simulink library "ammclib_bam_S32K3xx"  (R2016a)
(part 4 of 50)

      |     warning(['Parameter f16PropGain_Q of ' gcb ' exceeds the fixed-point range.']);
      |   end
      |   if f16PropGain_Q<-2^15
      |     f16PropGain_Q=-2^15;
      |     warning(['Parameter f16PropGain_Q of ' gcb ' exceeds the fixed-point range.']);
      |   end
      |   kifQ=igainQ*SampleTime*0.5*iscale/uscale;
      |   s16IntegGainShift_Q=ceil(log2(abs(kifQ)));
      |   if s16IntegGainShift_Q<-15
      |     s16IntegGainShift_Q=-15;
      |   end
      |   if s16IntegGainShift_Q>15
      |     s16IntegGainShift_Q=15;
      |     warning(['Parameter s16IntegGainShift_Q of ' gcb ' exceeds the fixed-point range.']);
      |   end
      |   f16IntegGain_Q=round(kifQ*2^(-s16IntegGainShift_Q)*2^15);
      |   if f16IntegGain_Q>2^15-1
      |     f16IntegGain_Q=2^15-1;
      |     warning(['Parameter f16IntegGain_Q of ' gcb ' exceeds the fixed-point range.']);
      |   end
      |   if f16IntegGain_Q<-2^15
      |     f16IntegGain_Q=-2^15;
      |     warning(['Parameter f16IntegGain_Q of ' gcb ' exceeds the fixed-point range.']);
      |   end
      |   if isnan(f16PropGain_D)
      |     if ~strcmp(f16PropGain_D_bkup,'0')
      |       set_param(gcb,'f16PropGain_D','0');
      |     end
      |   else
      |     tmps=num2str(f16PropGain_D);
      |     if ~strcmp(f16PropGain_D_bkup,tmps)
      |       set_param(gcb,'f16PropGain_D',tmps);
      |     end
      |   end
      |   if isnan(f16IntegGain_D)
      |     if ~strcmp(f16IntegGain_D_bkup,'0')
      |       set_param(gcb,'f16IntegGain_D','0');
      |     end
      |   else
      |     tmps=num2str(f16IntegGain_D);
      |     if ~strcmp(f16IntegGain_D_bkup,tmps)
      |       set_param(gcb,'f16IntegGain_D',tmps);
      |     end
      |   end
      |   if isnan(s16PropGainShift_D)
      |     if ~strcmp(s16PropGainShift_D_bkup,'0')
      |       set_param(gcb,'s16PropGainShift_D','0');
      |     end
      |   else
      |     tmps=num2str(s16PropGainShift_D);
      |     if ~strcmp(s16PropGainShift_D_bkup,tmps)
      |       set_param(gcb,'s16PropGainShift_D',tmps);
      |     end
      |   end
      |   if isnan(s16IntegGainShift_D)
      |     if ~strcmp(s16IntegGainShift_D_bkup,'0')
      |       set_param(gcb,'s16IntegGainShift_D','0');
      |     end
      |   else
      |     tmps=num2str(s16IntegGainShift_D);
      |     if ~strcmp(s16IntegGainShift_D_bkup,tmps)
      |       set_param(gcb,'s16IntegGainShift_D',tmps);
      |     end
      |   end
      |   if isnan(f16PropGain_Q)
      |     if ~strcmp(f16PropGain_Q_bkup,'0')
      |       set_param(gcb,'f16PropGain_Q','0');
      |     end
      |   else
      |     tmps=num2str(f16PropGain_Q);
      |     if ~strcmp(f16PropGain_Q_bkup,tmps)
      |       set_param(gcb,'f16PropGain_Q',tmps);
      |     end
      |   end
      |   if isnan(f16IntegGain_Q)
      |     if ~strcmp(f16IntegGain_Q_bkup,'0')
      |       set_param(gcb,'f16IntegGain_Q','0');
      |     end
      |   else
      |     tmps=num2str(f16IntegGain_Q);
      |     if ~strcmp(f16IntegGain_Q_bkup,tmps)
      |       set_param(gcb,'f16IntegGain_Q',tmps);
      |     end
      |   end
      |   if isnan(s16PropGainShift_Q)
      |     if ~strcmp(s16PropGainShift_Q_bkup,'0')
      |       set_param(gcb,'s16PropGainShift_Q','0');
      |     end
      |   else
      |     tmps=num2str(s16PropGainShift_Q);
      |     if ~strcmp(s16PropGainShift_Q_bkup,tmps)
      |       set_param(gcb,'s16PropGainShift_Q',tmps);
      |     end
      |   end
      |   if isnan(s16IntegGainShift_Q)
      |     if ~strcmp(s16IntegGainShift_Q_bkup,'0')
      |       set_param(gcb,'s16IntegGainShift_Q','0');
      |     end
      |   else
      |     tmps=num2str(s16IntegGainShift_Q);
      |     if ~strcmp(s16IntegGainShift_Q_bkup,tmps)
      |       set_param(gcb,'s16IntegGainShift_Q',tmps);
      |     end
      |   end
      | end
      mask Callback Lq:
      | autoCalcEn=get_param(gcb,'autoCalcEn');
      | if strcmp(autoCalcEn,'on')
      |   SampleTime=Simulink.data.evalinGlobal(bdroot,get_param(gcb,'SampleTime'));
      |   if (SampleTime==-1)
      |     SampleTime=str2double(get_param(gcb,'SampleTime_1'));
      |   end
      |   f16PropGain_D_bkup=get_param(gcb,'f16PropGain_D');
      |   f16IntegGain_D_bkup=get_param(gcb,'f16IntegGain_D');
      |   s16PropGainShift_D_bkup=get_param(gcb,'s16PropGainShift_D');
      |   s16IntegGainShift_D_bkup=get_param(gcb,'s16IntegGainShift_D');
      |   f16PropGain_Q_bkup=get_param(gcb,'f16PropGain_Q');
      |   f16IntegGain_Q_bkup=get_param(gcb,'f16IntegGain_Q');
      |   s16PropGainShift_Q_bkup=get_param(gcb,'s16PropGainShift_Q');
      |   s16IntegGainShift_Q_bkup=get_param(gcb,'s16IntegGainShift_Q');
      |   if0=Simulink.data.evalinGlobal(bdroot,get_param(gcb,'if0'));
      |   iksi=Simulink.data.evalinGlobal(bdroot,get_param(gcb,'iksi'));
      |   Ld=Simulink.data.evalinGlobal(bdroot,get_param(gcb,'Ld'));
      |   Lq=Simulink.data.evalinGlobal(bdroot,get_param(gcb,'Lq'));
      |   Rs=Simulink.data.evalinGlobal(bdroot,get_param(gcb,'Rs'));
      |   uscale=Simulink.data.evalinGlobal(bdroot,get_param(gcb,'uscale'));
      |   iscale=Simulink.data.evalinGlobal(bdroot,get_param(gcb,'iscale'));
      |   if (if0<=0)
      |     warning('Natural frequency f0 must be positive.');
      |   end
      |   if (iksi<=0)
      |     warning('Current loop attenuation must be positive.');
      |   end
      |   if (iksi>1)
      |     warning('Current loop attenuation must not exceed 1.');
      |   end
      |   if (Ld<=0)
      |     warning('Inductance Ld must be positive.');
      |   end
      |   if (Lq<=0)
      |     warning('Inductance Lq must be positive.');
      |   end
      |   if (Rs<0)
      |     warning('Resistance Rs must be non-negative.');
      |   end
      |   if (uscale<=0)
      |     warning('U_max must be positive.');
      |   end
      |   if (iscale<=0)
      |     warning('I_max must be positive.');
      |   end
      |   w0=6.283185307179586*if0;
      |   pgainD=2.0*iksi*w0*Ld-Rs;
      |   igainD=w0*w0*Ld;
      |   pgainQ=2.0*iksi*w0*Lq-Rs;
      |   igainQ=w0*w0*Lq;
      |   kpfD=pgainD*iscale/uscale;
      |   s16PropGainShift_D=ceil(log2(abs(kpfD)));
      |   if s16PropGainShift_D<-15
      |     s16PropGainShift_D=-15;
      |   end
      |   if s16PropGainShift_D>15
      |     s16PropGainShift_D=15;
      |     warning(['Parameter s16PropGainShift_D of ' gcb ' exceeds the fixed-point range.']);
      |   end
      |   f16PropGain_D=round(kpfD*2^(-s16PropGainShift_D)*2^15);
      |   if f16PropGain_D>2^15-1
      |     f16PropGain_D=2^15-1;
      |     warning(['Parameter f16PropGain_D of ' gcb ' exceeds the fixed-point range.']);
      |   end
      |   if f16PropGain_D<-2^15
      |     f16PropGain_D=-2^15;
      |     warning(['Parameter f16PropGain_D of ' gcb ' exceeds the fixed-point range.']);
      |   end
      |   kifD=igainD*SampleTime*0.5*iscale/uscale;
      |   s16IntegGainShift_D=ceil(log2(abs(kifD)));
      |   if s16IntegGainShift_D<-15
      |     s16IntegGainShift_D=-15;
      |   end
      |   if s16IntegGainShift_D>15
      |     s16IntegGainShift_D=15;
      |     warning(['Parameter s16IntegGainShift_D of ' gcb ' exceeds the fixed-point range.']);
      |   end
      |   f16IntegGain_D=round(kifD*2^(-s16IntegGainShift_D)*2^15);
      |   if f16IntegGain_D>2^15-1
      |     f16IntegGain_D=2^15-1;
      |     warning(['Parameter f16IntegGain_D of ' gcb ' exceeds the fixed-point range.']);
      |   end
      |   if f16IntegGain_D<-2^15
      |     f16IntegGain_D=-2^15;
      |     warning(['Parameter f16IntegGain_D of ' gcb ' exceeds the fixed-point range.']);
      |   end
      |   kpfQ=pgainQ*iscale/uscale;
      |   s16PropGainShift_Q=ceil(log2(abs(kpfQ)));
      |   if s16PropGainShift_Q<-15
      |     s16PropGainShift_Q=-15;
      |   end
      |   if s16PropGainShift_Q>15
      |     s16PropGainShift_Q=15;
      |     warning(['Parameter s16PropGainShift_Q of ' gcb ' exceeds the fixed-point range.']);
      |   end
      |   f16PropGain_Q=round(kpfQ*2^(-s16PropGainShift_Q)*2^15);
      |   if f16PropGain_Q>2^15-1
      |     f16PropGain_Q=2^15-1;
      |     warning(['Parameter f16PropGain_Q of ' gcb ' exceeds the fixed-point range.']);
      |   end
      |   if f16PropGain_Q<-2^15
      |     f16PropGain_Q=-2^15;
      |     warning(['Parameter f16PropGain_Q of ' gcb ' exceeds the fixed-point range.']);
      |   end
      |   kifQ=igainQ*SampleTime*0.5*iscale/uscale;
      |   s16IntegGainShift_Q=ceil(log2(abs(kifQ)));
      |   if s16IntegGainShift_Q<-15
      |     s16IntegGainShift_Q=-15;
      |   end
      |   if s16IntegGainShift_Q>15
      |     s16IntegGainShift_Q=15;
      |     warning(['Parameter s16IntegGainShift_Q of ' gcb ' exceeds the fixed-point range.']);
      |   end
      |   f16IntegGain_Q=round(kifQ*2^(-s16IntegGainShift_Q)*2^15);
      |   if f16IntegGain_Q>2^15-1
      |     f16IntegGain_Q=2^15-1;
      |     warning(['Parameter f16IntegGain_Q of ' gcb ' exceeds the fixed-point range.']);
      |   end
      |   if f16IntegGain_Q<-2^15
      |     f16IntegGain_Q=-2^15;
      |     warning(['Parameter f16IntegGain_Q of ' gcb ' exceeds the fixed-point range.']);
      |   end
      |   if isnan(f16PropGain_D)
      |     if ~strcmp(f16PropGain_D_bkup,'0')
      |       set_param(gcb,'f16PropGain_D','0');
      |     end
      |   else
      |     tmps=num2str(f16PropGain_D);
      |     if ~strcmp(f16PropGain_D_bkup,tmps)
      |       set_param(gcb,'f16PropGain_D',tmps);
      |     end
      |   end
      |   if isnan(f16IntegGain_D)
      |     if ~strcmp(f16IntegGain_D_bkup,'0')
      |       set_param(gcb,'f16IntegGain_D','0');
      |     end
      |   else
      |     tmps=num2str(f16IntegGain_D);
      |     if ~strcmp(f16IntegGain_D_bkup,tmps)
      |       set_param(gcb,'f16IntegGain_D',tmps);
      |     end
      |   end
      |   if isnan(s16PropGainShift_D)
      |     if ~strcmp(s16PropGainShift_D_bkup,'0')
      |       set_param(gcb,'s16PropGainShift_D','0');
      |     end
      |   else
      |     tmps=num2str(s16PropGainShift_D);
      |     if ~strcmp(s16PropGainShift_D_bkup,tmps)
      |       set_param(gcb,'s16PropGainShift_D',tmps);
      |     end
      |   end
      |   if isnan(s16IntegGainShift_D)
      |     if ~strcmp(s16IntegGainShift_D_bkup,'0')
      |       set_param(gcb,'s16IntegGainShift_D','0');
      |     end
      |   else
      |     tmps=num2str(s16IntegGainShift_D);
      |     if ~strcmp(s16IntegGainShift_D_bkup,tmps)
      |       set_param(gcb,'s16IntegGainShift_D',tmps);
      |     end
      |   end
      |   if isnan(f16PropGain_Q)
      |     if ~strcmp(f16PropGain_Q_bkup,'0')
      |       set_param(gcb,'f16PropGain_Q','0');
      |     end
      |   else
      |     tmps=num2str(f16PropGain_Q);
      |     if ~strcmp(f16PropGain_Q_bkup,tmps)
      |       set_param(gcb,'f16PropGain_Q',tmps);
      |     end
      |   end
      |   if isnan(f16IntegGain_Q)
      |     if ~strcmp(f16IntegGain_Q_bkup,'0')
      |       set_param(gcb,'f16IntegGain_Q','0');
      |     end
      |   else
      |     tmps=num2str(f16IntegGain_Q);
      |     if ~strcmp(f16IntegGain_Q_bkup,tmps)
      |       set_param(gcb,'f16IntegGain_Q',tmps);
      |     end
      |   end
      |   if isnan(s16PropGainShift_Q)
      |     if ~strcmp(s16PropGainShift_Q_bkup,'0')
      |       set_param(gcb,'s16PropGainShift_Q','0');
      |     end
      |   else
      |     tmps=num2str(s16PropGainShift_Q);
      |     if ~strcmp(s16PropGainShift_Q_bkup,tmps)
      |       set_param(gcb,'s16PropGainShift_Q',tmps);
      |     end
      |   end
      |   if isnan(s16IntegGainShift_Q)
      |     if ~strcmp(s16IntegGainShift_Q_bkup,'0')
      |       set_param(gcb,'s16IntegGainShift_Q','0');
      |     end
      |   else
      |     tmps=num2str(s16IntegGainShift_Q);
      |     if ~strcmp(s16IntegGainShift_Q_bkup,tmps)
      |       set_param(gcb,'s16IntegGainShift_Q',tmps);
      |     end
      |   end
      | end
      mask Callback Rs:
      | autoCalcEn=get_param(gcb,'autoCalcEn');
      | if strcmp(autoCalcEn,'on')
      |   SampleTime=Simulink.data.evalinGlobal(bdroot,get_param(gcb,'SampleTime'));
      |   if (SampleTime==-1)
      |     SampleTime=str2double(get_param(gcb,'SampleTime_1'));
      |   end
      |   f16PropGain_D_bkup=get_param(gcb,'f16PropGain_D');
      |   f16IntegGain_D_bkup=get_param(gcb,'f16IntegGain_D');
      |   s16PropGainShift_D_bkup=get_param(gcb,'s16PropGainShift_D');
      |   s16IntegGainShift_D_bkup=get_param(gcb,'s16IntegGainShift_D');
      |   f16PropGain_Q_bkup=get_param(gcb,'f16PropGain_Q');
      |   f16IntegGain_Q_bkup=get_param(gcb,'f16IntegGain_Q');
      |   s16PropGainShift_Q_bkup=get_param(gcb,'s16PropGainShift_Q');
      |   s16IntegGainShift_Q_bkup=get_param(gcb,'s16IntegGainShift_Q');
      |   if0=Simulink.data.evalinGlobal(bdroot,get_param(gcb,'if0'));
      |   iksi=Simulink.data.evalinGlobal(bdroot,get_param(gcb,'iksi'));
      |   Ld=Simulink.data.evalinGlobal(bdroot,get_param(gcb,'Ld'));
      |   Lq=Simulink.data.evalinGlobal(bdroot,get_param(gcb,'Lq'));
      |   Rs=Simulink.data.evalinGlobal(bdroot,get_param(gcb,'Rs'));
      |   uscale=Simulink.data.evalinGlobal(bdroot,get_param(gcb,'uscale'));
      |   iscale=Simulink.data.evalinGlobal(bdroot,get_param(gcb,'iscale'));
      |   if (if0<=0)
      |     warning('Natural frequency f0 must be positive.');
      |   end
      |   if (iksi<=0)
      |     warning('Current loop attenuation must be positive.');
      |   end
      |   if (iksi>1)
      |     warning('Current loop attenuation must not exceed 1.');
      |   end
      |   if (Ld<=0)
      |     warning('Inductance Ld must be positive.');
      |   end
      |   if (Lq<=0)
      |     warning('Inductance Lq must be positive.');
      |   end
      |   if (Rs<0)
      |     warning('Resistance Rs must be non-negative.');
      |   end
      |   if (uscale<=0)
      |     warning('U_max must be positive.');
      |   end
      |   if (iscale<=0)
      |     warning('I_max must be positive.');
      |   end
      |   w0=6.283185307179586*if0;
      |   pgainD=2.0*iksi*w0*Ld-Rs;
      |   igainD=w0*w0*Ld;
      |   pgainQ=2.0*iksi*w0*Lq-Rs;
      |   igainQ=w0*w0*Lq;
      |   kpfD=pgainD*iscale/uscale;
      |   s16PropGainShift_D=ceil(log2(abs(kpfD)));
      |   if s16PropGainShift_D<-15
      |     s16PropGainShift_D=-15;
      |   end
      |   if s16PropGainShift_D>15
      |     s16PropGainShift_D=15;
      |     warning(['Parameter s16PropGainShift_D of ' gcb ' exceeds the fixed-point range.']);
      |   end
      |   f16PropGain_D=round(kpfD*2^(-s16PropGainShift_D)*2^15);
      |   if f16PropGain_D>2^15-1
      |     f16PropGain_D=2^15-1;
      |     warning(['Parameter f16PropGain_D of ' gcb ' exceeds the fixed-point range.']);
      |   end
      |   if f16PropGain_D<-2^15
      |     f16PropGain_D=-2^15;
      |     warning(['Parameter f16PropGain_D of ' gcb ' exceeds the fixed-point range.']);
      |   end
      |   kifD=igainD*SampleTime*0.5*iscale/uscale;
      |   s16IntegGainShift_D=ceil(log2(abs(kifD)));
      |   if s16IntegGainShift_D<-15
      |     s16IntegGainShift_D=-15;
      |   end
      |   if s16IntegGainShift_D>15
      |     s16IntegGainShift_D=15;
      |     warning(['Parameter s16IntegGainShift_D of ' gcb ' exceeds the fixed-point range.']);
      |   end
      |   f16IntegGain_D=round(kifD*2^(-s16IntegGainShift_D)*2^15);
      |   if f16IntegGain_D>2^15-1
      |     f16IntegGain_D=2^15-1;
      |     warning(['Parameter f16IntegGain_D of ' gcb ' exceeds the fixed-point range.']);
      |   end
      |   if f16IntegGain_D<-2^15
      |     f16IntegGain_D=-2^15;
      |     warning(['Parameter f16IntegGain_D of ' gcb ' exceeds the fixed-point range.']);
      |   end
      |   kpfQ=pgainQ*iscale/uscale;
      |   s16PropGainShift_Q=ceil(log2(abs(kpfQ)));
      |   if s16PropGainShift_Q<-15
      |     s16PropGainShift_Q=-15;
      |   end
      |   if s16PropGainShift_Q>15
      |     s16PropGainShift_Q=15;
      |     warning(['Parameter s16PropGainShift_Q of ' gcb ' exceeds the fixed-point range.']);
      |   end
      |   f16PropGain_Q=round(kpfQ*2^(-s16PropGainShift_Q)*2^15);
      |   if f16PropGain_Q>2^15-1
      |     f16PropGain_Q=2^15-1;
      |     warning(['Parameter f16PropGain_Q of ' gcb ' exceeds the fixed-point range.']);
      |   end
      |   if f16PropGain_Q<-2^15
      |     f16PropGain_Q=-2^15;
      |     warning(['Parameter f16PropGain_Q of ' gcb ' exceeds the fixed-point range.']);
      |   end
      |   kifQ=igainQ*SampleTime*0.5*iscale/uscale;
      |   s16IntegGainShift_Q=ceil(log2(abs(kifQ)));
      |   if s16IntegGainShift_Q<-15
      |     s16IntegGainShift_Q=-15;
      |   end
      |   if s16IntegGainShift_Q>15
      |     s16IntegGainShift_Q=15;
      |     warning(['Parameter s16IntegGainShift_Q of ' gcb ' exceeds the fixed-point range.']);
      |   end
      |   f16IntegGain_Q=round(kifQ*2^(-s16IntegGainShift_Q)*2^15);
      |   if f16IntegGain_Q>2^15-1
      |     f16IntegGain_Q=2^15-1;
      |     warning(['Parameter f16IntegGain_Q of ' gcb ' exceeds the fixed-point range.']);
      |   end
      |   if f16IntegGain_Q<-2^15
      |     f16IntegGain_Q=-2^15;
      |     warning(['Parameter f16IntegGain_Q of ' gcb ' exceeds the fixed-point range.']);
      |   end
      |   if isnan(f16PropGain_D)
      |     if ~strcmp(f16PropGain_D_bkup,'0')
      |       set_param(gcb,'f16PropGain_D','0');
      |     end
      |   else
      |     tmps=num2str(f16PropGain_D);
      |     if ~strcmp(f16PropGain_D_bkup,tmps)
      |       set_param(gcb,'f16PropGain_D',tmps);
      |     end
      |   end
      |   if isnan(f16IntegGain_D)
      |     if ~strcmp(f16IntegGain_D_bkup,'0')
      |       set_param(gcb,'f16IntegGain_D','0');
      |     end
      |   else
      |     tmps=num2str(f16IntegGain_D);
      |     if ~strcmp(f16IntegGain_D_bkup,tmps)
      |       set_param(gcb,'f16IntegGain_D',tmps);
      |     end
      |   end
      |   if isnan(s16PropGainShift_D)
      |     if ~strcmp(s16PropGainShift_D_bkup,'0')
      |       set_param(gcb,'s16PropGainShift_D','0');
      |     end
      |   else
      |     tmps=num2str(s16PropGainShift_D);
      |     if ~strcmp(s16PropGainShift_D_bkup,tmps)
      |       set_param(gcb,'s16PropGainShift_D',tmps);
      |     end
      |   end
      |   if isnan(s16IntegGainShift_D)
      |     if ~strcmp(s16IntegGainShift_D_bkup,'0')
      |       set_param(gcb,'s16IntegGainShift_D','0');
      |     end
      |   else
      |     tmps=num2str(s16IntegGainShift_D);
      |     if ~strcmp(s16IntegGainShift_D_bkup,tmps)
      |       set_param(gcb,'s16IntegGainShift_D',tmps);
      |     end
      |   end
      |   if isnan(f16PropGain_Q)
      |     if ~strcmp(f16PropGain_Q_bkup,'0')
      |       set_param(gcb,'f16PropGain_Q','0');
      |     end
      |   else
      |     tmps=num2str(f16PropGain_Q);
      |     if ~strcmp(f16PropGain_Q_bkup,tmps)
      |       set_param(gcb,'f16PropGain_Q',tmps);
      |     end
      |   end
      |   if isnan(f16IntegGain_Q)
      |     if ~strcmp(f16IntegGain_Q_bkup,'0')
      |       set_param(gcb,'f16IntegGain_Q','0');
      |     end
      |   else
      |     tmps=num2str(f16IntegGain_Q);
      |     if ~strcmp(f16IntegGain_Q_bkup,tmps)
      |       set_param(gcb,'f16IntegGain_Q',tmps);
      |     end
      |   end
      |   if isnan(s16PropGainShift_Q)
      |     if ~strcmp(s16PropGainShift_Q_bkup,'0')
      |       set_param(gcb,'s16PropGainShift_Q','0');
      |     end
      |   else
      |     tmps=num2str(s16PropGainShift_Q);
      |     if ~strcmp(s16PropGainShift_Q_bkup,tmps)
      |       set_param(gcb,'s16PropGainShift_Q',tmps);
      |     end
      |   end
      |   if isnan(s16IntegGainShift_Q)
      |     if ~strcmp(s16IntegGainShift_Q_bkup,'0')
      |       set_param(gcb,'s16IntegGainShift_Q','0');
      |     end
      |   else
      |     tmps=num2str(s16IntegGainShift_Q);
      |     if ~strcmp(s16IntegGainShift_Q_bkup,tmps)
      |       set_param(gcb,'s16IntegGainShift_Q',tmps);
      |     end
      |   end
      | end
      mask Callback uscale:
      | autoCalcEn=get_param(gcb,'autoCalcEn');
      | if strcmp(autoCalcEn,'on')
      |   SampleTime=Simulink.data.evalinGlobal(bdroot,get_param(gcb,'SampleTime'));
      |   if (SampleTime==-1)
      |     SampleTime=str2double(get_param(gcb,'SampleTime_1'));
      |   end
      |   f16PropGain_D_bkup=get_param(gcb,'f16PropGain_D');
      |   f16IntegGain_D_bkup=get_param(gcb,'f16IntegGain_D');
      |   s16PropGainShift_D_bkup=get_param(gcb,'s16PropGainShift_D');
      |   s16IntegGainShift_D_bkup=get_param(gcb,'s16IntegGainShift_D');
      |   f16PropGain_Q_bkup=get_param(gcb,'f16PropGain_Q');
      |   f16IntegGain_Q_bkup=get_param(gcb,'f16IntegGain_Q');
      |   s16PropGainShift_Q_bkup=get_param(gcb,'s16PropGainShift_Q');
      |   s16IntegGainShift_Q_bkup=get_param(gcb,'s16IntegGainShift_Q');
      |   if0=Simulink.data.evalinGlobal(bdroot,get_param(gcb,'if0'));
      |   iksi=Simulink.data.evalinGlobal(bdroot,get_param(gcb,'iksi'));
      |   Ld=Simulink.data.evalinGlobal(bdroot,get_param(gcb,'Ld'));
      |   Lq=Simulink.data.evalinGlobal(bdroot,get_param(gcb,'Lq'));
      |   Rs=Simulink.data.evalinGlobal(bdroot,get_param(gcb,'Rs'));
      |   uscale=Simulink.data.evalinGlobal(bdroot,get_param(gcb,'uscale'));
      |   iscale=Simulink.data.evalinGlobal(bdroot,get_param(gcb,'iscale'));
      |   if (if0<=0)
      |     warning('Natural frequency f0 must be positive.');
      |   end
      |   if (iksi<=0)
      |     warning('Current loop attenuation must be positive.');
      |   end
      |   if (iksi>1)
      |     warning('Current loop attenuation must not exceed 1.');
      |   end
      |   if (Ld<=0)
      |     warning('Inductance Ld must be positive.');
      |   end
      |   if (Lq<=0)
      |     warning('Inductance Lq must be positive.');
      |   end
      |   if (Rs<0)
      |     warning('Resistance Rs must be non-negative.');
      |   end
      |   if (uscale<=0)
      |     warning('U_max must be positive.');
      |   end
      |   if (iscale<=0)
      |     warning('I_max must be positive.');
      |   end
      |   w0=6.283185307179586*if0;
      |   pgainD=2.0*iksi*w0*Ld-Rs;
      |   igainD=w0*w0*Ld;
      |   pgainQ=2.0*iksi*w0*Lq-Rs;
      |   igainQ=w0*w0*Lq;
      |   kpfD=pgainD*iscale/uscale;
      |   s16PropGainShift_D=ceil(log2(abs(kpfD)));
      |   if s16PropGainShift_D<-15
      |     s16PropGainShift_D=-15;
      |   end
      |   if s16PropGainShift_D>15
      |     s16PropGainShift_D=15;
      |     warning(['Parameter s16PropGainShift_D of ' gcb ' exceeds the fixed-point range.']);
      |   end
      |   f16PropGain_D=round(kpfD*2^(-s16PropGainShift_D)*2^15);
      |   if f16PropGain_D>2^15-1
      |     f16PropGain_D=2^15-1;
      |     warning(['Parameter f16PropGain_D of ' gcb ' exceeds the fixed-point range.']);
      |   end
      |   if f16PropGain_D<-2^15
      |     f16PropGain_D=-2^15;
      |     warning(['Parameter f16PropGain_D of ' gcb ' exceeds the fixed-point range.']);
      |   end
      |   kifD=igainD*SampleTime*0.5*iscale/uscale;
      |   s16IntegGainShift_D=ceil(log2(abs(kifD)));
      |   if s16IntegGainShift_D<-15
      |     s16IntegGainShift_D=-15;
      |   end
      |   if s16IntegGainShift_D>15
      |     s16IntegGainShift_D=15;
      |     warning(['Parameter s16IntegGainShift_D of ' gcb ' exceeds the fixed-point range.']);
      |   end
      |   f16IntegGain_D=round(kifD*2^(-s16IntegGainShift_D)*2^15);
      |   if f16IntegGain_D>2^15-1
      |     f16IntegGain_D=2^15-1;
      |     warning(['Parameter f16IntegGain_D of ' gcb ' exceeds the fixed-point range.']);
      |   end
      |   if f16IntegGain_D<-2^15
      |     f16IntegGain_D=-2^15;
      |     warning(['Parameter f16IntegGain_D of ' gcb ' exceeds the fixed-point range.']);
      |   end
      |   kpfQ=pgainQ*iscale/uscale;
      |   s16PropGainShift_Q=ceil(log2(abs(kpfQ)));
      |   if s16PropGainShift_Q<-15
      |     s16PropGainShift_Q=-15;
      |   end
      |   if s16PropGainShift_Q>15
      |     s16PropGainShift_Q=15;
      |     warning(['Parameter s16PropGainShift_Q of ' gcb ' exceeds the fixed-point range.']);
      |   end
      |   f16PropGain_Q=round(kpfQ*2^(-s16PropGainShift_Q)*2^15);
      |   if f16PropGain_Q>2^15-1
      |     f16PropGain_Q=2^15-1;
      |     warning(['Parameter f16PropGain_Q of ' gcb ' exceeds the fixed-point range.']);
      |   end
      |   if f16PropGain_Q<-2^15
      |     f16PropGain_Q=-2^15;
      |     warning(['Parameter f16PropGain_Q of ' gcb ' exceeds the fixed-point range.']);
      |   end
      |   kifQ=igainQ*SampleTime*0.5*iscale/uscale;
      |   s16IntegGainShift_Q=ceil(log2(abs(kifQ)));
      |   if s16IntegGainShift_Q<-15
      |     s16IntegGainShift_Q=-15;
      |   end
      |   if s16IntegGainShift_Q>15
      |     s16IntegGainShift_Q=15;
      |     warning(['Parameter s16IntegGainShift_Q of ' gcb ' exceeds the fixed-point range.']);
      |   end
      |   f16IntegGain_Q=round(kifQ*2^(-s16IntegGainShift_Q)*2^15);
      |   if f16IntegGain_Q>2^15-1
      |     f16IntegGain_Q=2^15-1;
      |     warning(['Parameter f16IntegGain_Q of ' gcb ' exceeds the fixed-point range.']);
      |   end
      |   if f16IntegGain_Q<-2^15
      |     f16IntegGain_Q=-2^15;
      |     warning(['Parameter f16IntegGain_Q of ' gcb ' exceeds the fixed-point range.']);
      |   end
      |   if isnan(f16PropGain_D)
      |     if ~strcmp(f16PropGain_D_bkup,'0')
      |       set_param(gcb,'f16PropGain_D','0');
      |     end
      |   else
      |     tmps=num2str(f16PropGain_D);
      |     if ~strcmp(f16PropGain_D_bkup,tmps)
      |       set_param(gcb,'f16PropGain_D',tmps);
      |     end
      |   end
      |   if isnan(f16IntegGain_D)
      |     if ~strcmp(f16IntegGain_D_bkup,'0')
      |       set_param(gcb,'f16IntegGain_D','0');
      |     end
      |   else
      |     tmps=num2str(f16IntegGain_D);
      |     if ~strcmp(f16IntegGain_D_bkup,tmps)
      |       set_param(gcb,'f16IntegGain_D',tmps);
      |     end
      |   end
      |   if isnan(s16PropGainShift_D)
      |     if ~strcmp(s16PropGainShift_D_bkup,'0')
      |       set_param(gcb,'s16PropGainShift_D','0');
      |     end
      |   else
      |     tmps=num2str(s16PropGainShift_D);
      |     if ~strcmp(s16PropGainShift_D_bkup,tmps)
      |       set_param(gcb,'s16PropGainShift_D',tmps);
      |     end
      |   end
      |   if isnan(s16IntegGainShift_D)
      |     if ~strcmp(s16IntegGainShift_D_bkup,'0')
      |       set_param(gcb,'s16IntegGainShift_D','0');
      |     end
      |   else
      |     tmps=num2str(s16IntegGainShift_D);
      |     if ~strcmp(s16IntegGainShift_D_bkup,tmps)
      |       set_param(gcb,'s16IntegGainShift_D',tmps);
      |     end
      |   end
      |   if isnan(f16PropGain_Q)
      |     if ~strcmp(f16PropGain_Q_bkup,'0')
      |       set_param(gcb,'f16PropGain_Q','0');
      |     end
      |   else
      |     tmps=num2str(f16PropGain_Q);
      |     if ~strcmp(f16PropGain_Q_bkup,tmps)
      |       set_param(gcb,'f16PropGain_Q',tmps);
      |     end
      |   end
      |   if isnan(f16IntegGain_Q)
      |     if ~strcmp(f16IntegGain_Q_bkup,'0')
      |       set_param(gcb,'f16IntegGain_Q','0');
      |     end
      |   else
      |     tmps=num2str(f16IntegGain_Q);
      |     if ~strcmp(f16IntegGain_Q_bkup,tmps)
      |       set_param(gcb,'f16IntegGain_Q',tmps);
      |     end
      |   end
      |   if isnan(s16PropGainShift_Q)
      |     if ~strcmp(s16PropGainShift_Q_bkup,'0')
      |       set_param(gcb,'s16PropGainShift_Q','0');
      |     end
      |   else
      |     tmps=num2str(s16PropGainShift_Q);
      |     if ~strcmp(s16PropGainShift_Q_bkup,tmps)
      |       set_param(gcb,'s16PropGainShift_Q',tmps);
      |     end
      |   end
      |   if isnan(s16IntegGainShift_Q)
      |     if ~strcmp(s16IntegGainShift_Q_bkup,'0')
      |       set_param(gcb,'s16IntegGainShift_Q','0');
      |     end
      |   else
      |     tmps=num2str(s16IntegGainShift_Q);
      |     if ~strcmp(s16IntegGainShift_Q_bkup,tmps)
      |       set_param(gcb,'s16IntegGainShift_Q',tmps);
      |     end
      |   end
      | end
      mask Callback iscale:
      | autoCalcEn=get_param(gcb,'autoCalcEn');
      | if strcmp(autoCalcEn,'on')
      |   SampleTime=Simulink.data.evalinGlobal(bdroot,get_param(gcb,'SampleTime'));
      |   if (SampleTime==-1)
      |     SampleTime=str2double(get_param(gcb,'SampleTime_1'));
      |   end
      |   f16PropGain_D_bkup=get_param(gcb,'f16PropGain_D');
      |   f16IntegGain_D_bkup=get_param(gcb,'f16IntegGain_D');
      |   s16PropGainShift_D_bkup=get_param(gcb,'s16PropGainShift_D');
      |   s16IntegGainShift_D_bkup=get_param(gcb,'s16IntegGainShift_D');
      |   f16PropGain_Q_bkup=get_param(gcb,'f16PropGain_Q');
      |   f16IntegGain_Q_bkup=get_param(gcb,'f16IntegGain_Q');
      |   s16PropGainShift_Q_bkup=get_param(gcb,'s16PropGainShift_Q');
      |   s16IntegGainShift_Q_bkup=get_param(gcb,'s16IntegGainShift_Q');
      |   if0=Simulink.data.evalinGlobal(bdroot,get_param(gcb,'if0'));
      |   iksi=Simulink.data.evalinGlobal(bdroot,get_param(gcb,'iksi'));
      |   Ld=Simulink.data.evalinGlobal(bdroot,get_param(gcb,'Ld'));
      |   Lq=Simulink.data.evalinGlobal(bdroot,get_param(gcb,'Lq'));
      |   Rs=Simulink.data.evalinGlobal(bdroot,get_param(gcb,'Rs'));
      |   uscale=Simulink.data.evalinGlobal(bdroot,get_param(gcb,'uscale'));
      |   iscale=Simulink.data.evalinGlobal(bdroot,get_param(gcb,'iscale'));
      |   if (if0<=0)
      |     warning('Natural frequency f0 must be positive.');
      |   end
      |   if (iksi<=0)
      |     warning('Current loop attenuation must be positive.');
      |   end
      |   if (iksi>1)
      |     warning('Current loop attenuation must not exceed 1.');
      |   end
      |   if (Ld<=0)
      |     warning('Inductance Ld must be positive.');
      |   end
      |   if (Lq<=0)
      |     warning('Inductance Lq must be positive.');
      |   end
      |   if (Rs<0)
      |     warning('Resistance Rs must be non-negative.');
      |   end
      |   if (uscale<=0)
      |     warning('U_max must be positive.');
      |   end
      |   if (iscale<=0)
      |     warning('I_max must be positive.');
      |   end
      |   w0=6.283185307179586*if0;
      |   pgainD=2.0*iksi*w0*Ld-Rs;
      |   igainD=w0*w0*Ld;
      |   pgainQ=2.0*iksi*w0*Lq-Rs;
      |   igainQ=w0*w0*Lq;
      |   kpfD=pgainD*iscale/uscale;
      |   s16PropGainShift_D=ceil(log2(abs(kpfD)));
      |   if s16PropGainShift_D<-15
      |     s16PropGainShift_D=-15;
      |   end
      |   if s16PropGainShift_D>15
      |     s16PropGainShift_D=15;
      |     warning(['Parameter s16PropGainShift_D of ' gcb ' exceeds the fixed-point range.']);
      |   end
      |   f16PropGain_D=round(kpfD*2^(-s16PropGainShift_D)*2^15);
      |   if f16PropGain_D>2^15-1
      |     f16PropGain_D=2^15-1;
      |     warning(['Parameter f16PropGain_D of ' gcb ' exceeds the fixed-point range.']);
      |   end
      |   if f16PropGain_D<-2^15
      |     f16PropGain_D=-2^15;
      |     warning(['Parameter f16PropGain_D of ' gcb ' exceeds the fixed-point range.']);
      |   end
      |   kifD=igainD*SampleTime*0.5*iscale/uscale;
      |   s16IntegGainShift_D=ceil(log2(abs(kifD)));
      |   if s16IntegGainShift_D<-15
      |     s16IntegGainShift_D=-15;
      |   end
      |   if s16IntegGainShift_D>15
      |     s16IntegGainShift_D=15;
      |     warning(['Parameter s16IntegGainShift_D of ' gcb ' exceeds the fixed-point range.']);
      |   end
      |   f16IntegGain_D=round(kifD*2^(-s16IntegGainShift_D)*2^15);
      |   if f16IntegGain_D>2^15-1
      |     f16IntegGain_D=2^15-1;
      |     warning(['Parameter f16IntegGain_D of ' gcb ' exceeds the fixed-point range.']);
      |   end
      |   if f16IntegGain_D<-2^15
      |     f16IntegGain_D=-2^15;
      |     warning(['Parameter f16IntegGain_D of ' gcb ' exceeds the fixed-point range.']);
      |   end
      |   kpfQ=pgainQ*iscale/uscale;
      |   s16PropGainShift_Q=ceil(log2(abs(kpfQ)));
      |   if s16PropGainShift_Q<-15
      |     s16PropGainShift_Q=-15;
      |   end
      |   if s16PropGainShift_Q>15
      |     s16PropGainShift_Q=15;
      |     warning(['Parameter s16PropGainShift_Q of ' gcb ' exceeds the fixed-point range.']);
      |   end
      |   f16PropGain_Q=round(kpfQ*2^(-s16PropGainShift_Q)*2^15);
      |   if f16PropGain_Q>2^15-1
      |     f16PropGain_Q=2^15-1;
      |     warning(['Parameter f16PropGain_Q of ' gcb ' exceeds the fixed-point range.']);
      |   end
      |   if f16PropGain_Q<-2^15
      |     f16PropGain_Q=-2^15;
      |     warning(['Parameter f16PropGain_Q of ' gcb ' exceeds the fixed-point range.']);
      |   end
      |   kifQ=igainQ*SampleTime*0.5*iscale/uscale;
      |   s16IntegGainShift_Q=ceil(log2(abs(kifQ)));
      |   if s16IntegGainShift_Q<-15
      |     s16IntegGainShift_Q=-15;
      |   end
      |   if s16IntegGainShift_Q>15
      |     s16IntegGainShift_Q=15;
      |     warning(['Parameter s16IntegGainShift_Q of ' gcb ' exceeds the fixed-point range.']);
      |   end
      |   f16IntegGain_Q=round(kifQ*2^(-s16IntegGainShift_Q)*2^15);
      |   if f16IntegGain_Q>2^15-1
      |     f16IntegGain_Q=2^15-1;
      |     warning(['Parameter f16IntegGain_Q of ' gcb ' exceeds the fixed-point range.']);
      |   end
      |   if f16IntegGain_Q<-2^15
      |     f16IntegGain_Q=-2^15;
      |     warning(['Parameter f16IntegGain_Q of ' gcb ' exceeds the fixed-point range.']);
      |   end
      |   if isnan(f16PropGain_D)
      |     if ~strcmp(f16PropGain_D_bkup,'0')
      |       set_param(gcb,'f16PropGain_D','0');
      |     end
      |   else
      |     tmps=num2str(f16PropGain_D);
      |     if ~strcmp(f16PropGain_D_bkup,tmps)
      |       set_param(gcb,'f16PropGain_D',tmps);
      |     end
      |   end
      |   if isnan(f16IntegGain_D)
      |     if ~strcmp(f16IntegGain_D_bkup,'0')
      |       set_param(gcb,'f16IntegGain_D','0');
      |     end
      |   else
      |     tmps=num2str(f16IntegGain_D);
      |     if ~strcmp(f16IntegGain_D_bkup,tmps)
      |       set_param(gcb,'f16IntegGain_D',tmps);
      |     end
      |   end
      |   if isnan(s16PropGainShift_D)
      |     if ~strcmp(s16PropGainShift_D_bkup,'0')
      |       set_param(gcb,'s16PropGainShift_D','0');
      |     end
      |   else
      |     tmps=num2str(s16PropGainShift_D);
      |     if ~strcmp(s16PropGainShift_D_bkup,tmps)
      |       set_param(gcb,'s16PropGainShift_D',tmps);
      |     end
      |   end
      |   if isnan(s16IntegGainShift_D)
      |     if ~strcmp(s16IntegGainShift_D_bkup,'0')
      |       set_param(gcb,'s16IntegGainShift_D','0');
      |     end
      |   else
      |     tmps=num2str(s16IntegGainShift_D);
      |     if ~strcmp(s16IntegGainShift_D_bkup,tmps)
      |       set_param(gcb,'s16IntegGainShift_D',tmps);
      |     end
      |   end
      |   if isnan(f16PropGain_Q)
      |     if ~strcmp(f16PropGain_Q_bkup,'0')
      |       set_param(gcb,'f16PropGain_Q','0');
      |     end
      |   else
      |     tmps=num2str(f16PropGain_Q);
      |     if ~strcmp(f16PropGain_Q_bkup,tmps)
      |       set_param(gcb,'f16PropGain_Q',tmps);
      |     end
      |   end
      |   if isnan(f16IntegGain_Q)
      |     if ~strcmp(f16IntegGain_Q_bkup,'0')
      |       set_param(gcb,'f16IntegGain_Q','0');
      |     end
      |   else
      |     tmps=num2str(f16IntegGain_Q);
      |     if ~strcmp(f16IntegGain_Q_bkup,tmps)
      |       set_param(gcb,'f16IntegGain_Q',tmps);
      |     end
      |   end
      |   if isnan(s16PropGainShift_Q)
      |     if ~strcmp(s16PropGainShift_Q_bkup,'0')
      |       set_param(gcb,'s16PropGainShift_Q','0');
      |     end
      |   else
      |     tmps=num2str(s16PropGainShift_Q);
      |     if ~strcmp(s16PropGainShift_Q_bkup,tmps)
      |       set_param(gcb,'s16PropGainShift_Q',tmps);
      |     end
      |   end
      |   if isnan(s16IntegGainShift_Q)
      |     if ~strcmp(s16IntegGainShift_Q_bkup,'0')
      |       set_param(gcb,'s16IntegGainShift_Q','0');
      |     end
      |   else
      |     tmps=num2str(s16IntegGainShift_Q);
      |     if ~strcmp(s16IntegGainShift_Q_bkup,tmps)
      |       set_param(gcb,'s16IntegGainShift_Q',tmps);
      |     end
      |   end
      | end
      mask Callback autoCalcEn:
      | maskStr=get_param(gcb,'showStates');
      | if strcmp(maskStr,'Hide (faster execution)')
      |   p=Simulink.Mask.get(gcb);
      |   autoCalcEn=get_param(gcb,'autoCalcEn');
      |   hintText=p.getDialogControl('timeHint');
      |   if strcmp(autoCalcEn,'on')
      |     param=p.getParameter('iscale');
      |     if strcmp(param.Enabled,'off')
      |       SampleTime=Simulink.data.evalinGlobal(bdroot,get_param(gcb,'SampleTime'));
      |       if SampleTime==-1
      |         SampleTime=str2double(get_param(gcb,'SampleTime_1'));
      |         if isnan(SampleTime)
      |           hintText.Prompt=['Note: Implementation parameters cannot be calculated yet because the block''s inherited sample time is unknown. Simulink will update the sample time when you run the simulation.'];
      |         else
      |           hintText.Prompt=['Caution: Implementation parameters depend on inherited sample time. Make sure that the sample time of the block''s inputs corresponds to the sampling period in the target application.'];
      |         end
      |       else
      |         hintText.Prompt='Caution: Implementation parameters depend on the sample time. Make sure that the simulation time step corresponds to the sampling period in the target application.';
      |       end
      |       p=Simulink.Mask.get(gcb);
      |       param=p.getParameter('if0');
      |       param.set('Enabled','on');
      |       param=p.getParameter('iksi');
      |       param.set('Enabled','on');
      |       param=p.getParameter('Ld');
      |       param.set('Enabled','on');
      |       param=p.getParameter('Lq');
      |       param.set('Enabled','on');
      |       param=p.getParameter('Rs');
      |       param.set('Enabled','on');
      |       param=p.getParameter('uscale');
      |       param.set('Enabled','on');
      |       param=p.getParameter('iscale');
      |       param.set('Enabled','on');
      |     else
      |       SampleTime=Simulink.data.evalinGlobal(bdroot,get_param(gcb,'SampleTime'));
      |       if SampleTime==-1
      |         SampleTime=str2double(get_param(gcb,'SampleTime_1'));
      |       end
      |     end
      |     f16PropGain_D_bkup=get_param(gcb,'f16PropGain_D');
      |     f16IntegGain_D_bkup=get_param(gcb,'f16IntegGain_D');
      |     s16PropGainShift_D_bkup=get_param(gcb,'s16PropGainShift_D');
      |     s16IntegGainShift_D_bkup=get_param(gcb,'s16IntegGainShift_D');
      |     f16PropGain_Q_bkup=get_param(gcb,'f16PropGain_Q');
      |     f16IntegGain_Q_bkup=get_param(gcb,'f16IntegGain_Q');
      |     s16PropGainShift_Q_bkup=get_param(gcb,'s16PropGainShift_Q');
      |     s16IntegGainShift_Q_bkup=get_param(gcb,'s16IntegGainShift_Q');
      |     if0=Simulink.data.evalinGlobal(bdroot,get_param(gcb,'if0'));
      |     iksi=Simulink.data.evalinGlobal(bdroot,get_param(gcb,'iksi'));
      |     Ld=Simulink.data.evalinGlobal(bdroot,get_param(gcb,'Ld'));
      |     Lq=Simulink.data.evalinGlobal(bdroot,get_param(gcb,'Lq'));
      |     Rs=Simulink.data.evalinGlobal(bdroot,get_param(gcb,'Rs'));
      |     uscale=Simulink.data.evalinGlobal(bdroot,get_param(gcb,'uscale'));
      |     iscale=Simulink.data.evalinGlobal(bdroot,get_param(gcb,'iscale'));
      |     if (if0<=0)
      |       warning('Natural frequency f0 must be positive.');
      |     end
      |     if (iksi<=0)
      |       warning('Current loop attenuation must be positive.');
      |     end
      |     if (iksi>1)
      |       warning('Current loop attenuation must not exceed 1.');
      |     end
      |     if (Ld<=0)
      |       warning('Inductance Ld must be positive.');
      |     end
      |     if (Lq<=0)
      |       warning('Inductance Lq must be positive.');
      |     end
      |     if (Rs<0)
      |       warning('Resistance Rs must be non-negative.');
      |     end
      |     if (uscale<=0)
      |       warning('U_max must be positive.');
      |     end
      |     if (iscale<=0)
      |       warning('I_max must be positive.');
      |     end
      |     w0=6.283185307179586*if0;
      |     pgainD=2.0*iksi*w0*Ld-Rs;
      |     igainD=w0*w0*Ld;
      |     pgainQ=2.0*iksi*w0*Lq-Rs;
      |     igainQ=w0*w0*Lq;
      |     kpfD=pgainD*iscale/uscale;
      |     s16PropGainShift_D=ceil(log2(abs(kpfD)));
      |     if s16PropGainShift_D<-15
      |       s16PropGainShift_D=-15;
      |     end
      |     if s16PropGainShift_D>15
      |       s16PropGainShift_D=15;
      |       warning(['Parameter s16PropGainShift_D of ' gcb ' exceeds the fixed-point range.']);
      |     end
      |     f16PropGain_D=round(kpfD*2^(-s16PropGainShift_D)*2^15);
      |     if f16PropGain_D>2^15-1
      |       f16PropGain_D=2^15-1;
      |       warning(['Parameter f16PropGain_D of ' gcb ' exceeds the fixed-point range.']);
      |     end
      |     if f16PropGain_D<-2^15
      |       f16PropGain_D=-2^15;
      |       warning(['Parameter f16PropGain_D of ' gcb ' exceeds the fixed-point range.']);
      |     end
      |     kifD=igainD*SampleTime*0.5*iscale/uscale;
      |     s16IntegGainShift_D=ceil(log2(abs(kifD)));
      |     if s16IntegGainShift_D<-15
      |       s16IntegGainShift_D=-15;
      |     end
      |     if s16IntegGainShift_D>15
      |       s16IntegGainShift_D=15;
      |       warning(['Parameter s16IntegGainShift_D of ' gcb ' exceeds the fixed-point range.']);
      |     end
      |     f16IntegGain_D=round(kifD*2^(-s16IntegGainShift_D)*2^15);
      |     if f16IntegGain_D>2^15-1
      |       f16IntegGain_D=2^15-1;
      |       warning(['Parameter f16IntegGain_D of ' gcb ' exceeds the fixed-point range.']);
      |     end
      |     if f16IntegGain_D<-2^15
      |       f16IntegGain_D=-2^15;
      |       warning(['Parameter f16IntegGain_D of ' gcb ' exceeds the fixed-point range.']);
      |     end
      |     kpfQ=pgainQ*iscale/uscale;
      |     s16PropGainShift_Q=ceil(log2(abs(kpfQ)));
      |     if s16PropGainShift_Q<-15
      |       s16PropGainShift_Q=-15;
      |     end
      |     if s16PropGainShift_Q>15
      |       s16PropGainShift_Q=15;
      |       warning(['Parameter s16PropGainShift_Q of ' gcb ' exceeds the fixed-point range.']);
      |     end
      |     f16PropGain_Q=round(kpfQ*2^(-s16PropGainShift_Q)*2^15);
      |     if f16PropGain_Q>2^15-1
      |       f16PropGain_Q=2^15-1;
      |       warning(['Parameter f16PropGain_Q of ' gcb ' exceeds the fixed-point range.']);
      |     end
      |     if f16PropGain_Q<-2^15
      |       f16PropGain_Q=-2^15;
      |       warning(['Parameter f16PropGain_Q of ' gcb ' exceeds the fixed-point range.']);
      |     end
      |     kifQ=igainQ*SampleTime*0.5*iscale/uscale;
      |     s16IntegGainShift_Q=ceil(log2(abs(kifQ)));
      |     if s16IntegGainShift_Q<-15
      |       s16IntegGainShift_Q=-15;
      |     end
      |     if s16IntegGainShift_Q>15
      |       s16IntegGainShift_Q=15;
      |       warning(['Parameter s16IntegGainShift_Q of ' gcb ' exceeds the fixed-point range.']);
      |     end
      |     f16IntegGain_Q=round(kifQ*2^(-s16IntegGainShift_Q)*2^15);
      |     if f16IntegGain_Q>2^15-1
      |       f16IntegGain_Q=2^15-1;
      |       warning(['Parameter f16IntegGain_Q of ' gcb ' exceeds the fixed-point range.']);
      |     end
      |     if f16IntegGain_Q<-2^15
      |       f16IntegGain_Q=-2^15;
      |       warning(['Parameter f16IntegGain_Q of ' gcb ' exceeds the fixed-point range.']);
      |     end
      |     if isnan(f16PropGain_D)
      |       if ~strcmp(f16PropGain_D_bkup,'0')
      |         set_param(gcb,'f16PropGain_D','0');
      |       end
      |     else
      |       tmps=num2str(f16PropGain_D);
      |       if ~strcmp(f16PropGain_D_bkup,tmps)
      |         set_param(gcb,'f16PropGain_D',tmps);
      |       end
      |     end
      |     if isnan(f16IntegGain_D)
      |       if ~strcmp(f16IntegGain_D_bkup,'0')
      |         set_param(gcb,'f16IntegGain_D','0');
      |       end
      |     else
      |       tmps=num2str(f16IntegGain_D);
      |       if ~strcmp(f16IntegGain_D_bkup,tmps)
      |         set_param(gcb,'f16IntegGain_D',tmps);
      |       end
      |     end
      |     if isnan(s16PropGainShift_D)
      |       if ~strcmp(s16PropGainShift_D_bkup,'0')
      |         set_param(gcb,'s16PropGainShift_D','0');
      |       end
      |     else
      |       tmps=num2str(s16PropGainShift_D);
      |       if ~strcmp(s16PropGainShift_D_bkup,tmps)
      |         set_param(gcb,'s16PropGainShift_D',tmps);
      |       end
      |     end
      |     if isnan(s16IntegGainShift_D)
      |       if ~strcmp(s16IntegGainShift_D_bkup,'0')
      |         set_param(gcb,'s16IntegGainShift_D','0');
      |       end
      |     else
      |       tmps=num2str(s16IntegGainShift_D);
      |       if ~strcmp(s16IntegGainShift_D_bkup,tmps)
      |         set_param(gcb,'s16IntegGainShift_D',tmps);
      |       end
      |     end
      |     if isnan(f16PropGain_Q)
      |       if ~strcmp(f16PropGain_Q_bkup,'0')
      |         set_param(gcb,'f16PropGain_Q','0');
      |       end
      |     else
      |       tmps=num2str(f16PropGain_Q);
      |       if ~strcmp(f16PropGain_Q_bkup,tmps)
      |         set_param(gcb,'f16PropGain_Q',tmps);
      |       end
      |     end
      |     if isnan(f16IntegGain_Q)
      |       if ~strcmp(f16IntegGain_Q_bkup,'0')
      |         set_param(gcb,'f16IntegGain_Q','0');
      |       end
      |     else
      |       tmps=num2str(f16IntegGain_Q);
      |       if ~strcmp(f16IntegGain_Q_bkup,tmps)
      |         set_param(gcb,'f16IntegGain_Q',tmps);
      |       end
      |     end
      |     if isnan(s16PropGainShift_Q)
      |       if ~strcmp(s16PropGainShift_Q_bkup,'0')
      |         set_param(gcb,'s16PropGainShift_Q','0');
      |       end
      |     else
      |       tmps=num2str(s16PropGainShift_Q);
      |       if ~strcmp(s16PropGainShift_Q_bkup,tmps)
      |         set_param(gcb,'s16PropGainShift_Q',tmps);
      |       end
      |     end
      |     if isnan(s16IntegGainShift_Q)
      |       if ~strcmp(s16IntegGainShift_Q_bkup,'0')
      |         set_param(gcb,'s16IntegGainShift_Q','0');
      |       end
      |     else
      |       tmps=num2str(s16IntegGainShift_Q);
      |       if ~strcmp(s16IntegGainShift_Q_bkup,tmps)
      |         set_param(gcb,'s16IntegGainShift_Q',tmps);
      |       end
      |     end
      |   else
      |     param=p.getParameter('iscale');
      |     if strcmp(param.Enabled,'on')
      |       hintText.Prompt='Caution: Implementation parameters are fixed.';
      |       p=Simulink.Mask.get(gcb);
      |       param=p.getParameter('if0');
      |       param.set('Enabled','off');
      |       param=p.getParameter('iksi');
      |       param.set('Enabled','off');
      |       param=p.getParameter('Ld');
      |       param.set('Enabled','off');
      |       param=p.getParameter('Lq');
      |       param.set('Enabled','off');
      |       param=p.getParameter('Rs');
      |       param.set('Enabled','off');
      |       param=p.getParameter('uscale');
      |       param.set('Enabled','off');
      |       param=p.getParameter('iscale');
      |       param.set('Enabled','off');
      |     end
      |   end
      | end
      mask DialogControl CompBut Prompt: Recalculate sample times
      mask DialogControl CompBut Tooltip: Simulink updates the sample times of all blocks when the simulation is run. This button will update the sample times now.
      mask DialogControl CompBut Callback:
      | btn=questdlg('This will apply all changes in all open dialog boxes and update the schematic. Do you want to proceed?','Apply all changes','Continue','Cancel','Continue');
      | if strcmp(btn,'Continue')
      |   dlgs=DAStudio.ToolRoot.getOpenDialogs;
      |   for i=1:length(dlgs)
      |     dlgs(i).apply;
      |   end
      |   try
      |     SampleTime_1=str2double(get_param(gcb,'SampleTime_1'));
      |     ts=Simulink.Block.getSampleTimes(gcb);
      |     ts=ts(1).Value(1);
      |     if (SampleTime_1 ~= ts)
      |       SampleTime_1=ts;
      |       set_param(gcb,'SampleTime_1',num2str(ts));
      |       autoCalcEn=get_param(gcb,'autoCalcEn');
      |       if strcmp(autoCalcEn,'on')
      |         SampleTime=Simulink.data.evalinGlobal(bdroot,get_param(gcb,'SampleTime'));
      |         p=Simulink.Mask.get(gcb);
      |         hintText=p.getDialogControl('timeHint');
      |         if SampleTime==-1
      |           SampleTime=SampleTime_1;
      |           hintText.Prompt='Caution: Implementation parameters depend on inherited sample time. Make sure that the sample time of the block''s inputs corresponds to the sampling period in the target application.';
      |         else
      |           hintText.Prompt='Caution: Implementation parameters depend on the sample time. Make sure that the simulation time step corresponds to the sampling period in the target application.';
      |         end
      |         f16PropGain_D_bkup=get_param(gcb,'f16PropGain_D');
      |         f16IntegGain_D_bkup=get_param(gcb,'f16IntegGain_D');
      |         s16PropGainShift_D_bkup=get_param(gcb,'s16PropGainShift_D');
      |         s16IntegGainShift_D_bkup=get_param(gcb,'s16IntegGainShift_D');
      |         f16PropGain_Q_bkup=get_param(gcb,'f16PropGain_Q');
      |         f16IntegGain_Q_bkup=get_param(gcb,'f16IntegGain_Q');
      |         s16PropGainShift_Q_bkup=get_param(gcb,'s16PropGainShift_Q');
      |         s16IntegGainShift_Q_bkup=get_param(gcb,'s16IntegGainShift_Q');
      |         if0=Simulink.data.evalinGlobal(bdroot,get_param(gcb,'if0'));
      |         iksi=Simulink.data.evalinGlobal(bdroot,get_param(gcb,'iksi'));
      |         Ld=Simulink.data.evalinGlobal(bdroot,get_param(gcb,'Ld'));
      |         Lq=Simulink.data.evalinGlobal(bdroot,get_param(gcb,'Lq'));
      |         Rs=Simulink.data.evalinGlobal(bdroot,get_param(gcb,'Rs'));
      |         uscale=Simulink.data.evalinGlobal(bdroot,get_param(gcb,'uscale'));
      |         iscale=Simulink.data.evalinGlobal(bdroot,get_param(gcb,'iscale'));
      |         if (if0<=0)
      |           warning('Natural frequency f0 must be positive.');
      |         end
      |         if (iksi<=0)
      |           warning('Current loop attenuation must be positive.');
      |         end
      |         if (iksi>1)
      |           warning('Current loop attenuation must not exceed 1.');
      |         end
      |         if (Ld<=0)
      |           warning('Inductance Ld must be positive.');
      |         end
      |         if (Lq<=0)
      |           warning('Inductance Lq must be positive.');
      |         end
      |         if (Rs<0)
      |           warning('Resistance Rs must be non-negative.');
      |         end
      |         if (uscale<=0)
      |           warning('U_max must be positive.');
      |         end
      |         if (iscale<=0)
      |           warning('I_max must be positive.');
      |         end
      |         w0=6.283185307179586*if0;
      |         pgainD=2.0*iksi*w0*Ld-Rs;
      |         igainD=w0*w0*Ld;
      |         pgainQ=2.0*iksi*w0*Lq-Rs;
      |         igainQ=w0*w0*Lq;
      |         kpfD=pgainD*iscale/uscale;
      |         s16PropGainShift_D=ceil(log2(abs(kpfD)));
      |         if s16PropGainShift_D<-15
      |           s16PropGainShift_D=-15;
      |         end
      |         if s16PropGainShift_D>15
      |           s16PropGainShift_D=15;
      |           warning(['Parameter s16PropGainShift_D of ' gcb ' exceeds the fixed-point range.']);
      |         end
      |         f16PropGain_D=round(kpfD*2^(-s16PropGainShift_D)*2^15);
      |         if f16PropGain_D>2^15-1
      |           f16PropGain_D=2^15-1;
      |           warning(['Parameter f16PropGain_D of ' gcb ' exceeds the fixed-point range.']);
      |         end
      |         if f16PropGain_D<-2^15
      |           f16PropGain_D=-2^15;
      |           warning(['Parameter f16PropGain_D of ' gcb ' exceeds the fixed-point range.']);
      |         end
      |         kifD=igainD*SampleTime*0.5*iscale/uscale;
      |         s16IntegGainShift_D=ceil(log2(abs(kifD)));
      |         if s16IntegGainShift_D<-15
      |           s16IntegGainShift_D=-15;
      |         end
      |         if s16IntegGainShift_D>15
      |           s16IntegGainShift_D=15;
      |           warning(['Parameter s16IntegGainShift_D of ' gcb ' exceeds the fixed-point range.']);
      |         end
      |         f16IntegGain_D=round(kifD*2^(-s16IntegGainShift_D)*2^15);
      |         if f16IntegGain_D>2^15-1
      |           f16IntegGain_D=2^15-1;
      |           warning(['Parameter f16IntegGain_D of ' gcb ' exceeds the fixed-point range.']);
      |         end
      |         if f16IntegGain_D<-2^15
      |           f16IntegGain_D=-2^15;
      |           warning(['Parameter f16IntegGain_D of ' gcb ' exceeds the fixed-point range.']);
      |         end
      |         kpfQ=pgainQ*iscale/uscale;
      |         s16PropGainShift_Q=ceil(log2(abs(kpfQ)));
      |         if s16PropGainShift_Q<-15
      |           s16PropGainShift_Q=-15;
      |         end
      |         if s16PropGainShift_Q>15
      |           s16PropGainShift_Q=15;
      |           warning(['Parameter s16PropGainShift_Q of ' gcb ' exceeds the fixed-point range.']);
      |         end
      |         f16PropGain_Q=round(kpfQ*2^(-s16PropGainShift_Q)*2^15);
      |         if f16PropGain_Q>2^15-1
      |           f16PropGain_Q=2^15-1;
      |           warning(['Parameter f16PropGain_Q of ' gcb ' exceeds the fixed-point range.']);
      |         end
      |         if f16PropGain_Q<-2^15
      |           f16PropGain_Q=-2^15;
      |           warning(['Parameter f16PropGain_Q of ' gcb ' exceeds the fixed-point range.']);
      |         end
      |         kifQ=igainQ*SampleTime*0.5*iscale/uscale;
      |         s16IntegGainShift_Q=ceil(log2(abs(kifQ)));
      |         if s16IntegGainShift_Q<-15
      |           s16IntegGainShift_Q=-15;
      |         end
      |         if s16IntegGainShift_Q>15
      |           s16IntegGainShift_Q=15;
      |           warning(['Parameter s16IntegGainShift_Q of ' gcb ' exceeds the fixed-point range.']);
      |         end
      |         f16IntegGain_Q=round(kifQ*2^(-s16IntegGainShift_Q)*2^15);
      |         if f16IntegGain_Q>2^15-1
      |           f16IntegGain_Q=2^15-1;
      |           warning(['Parameter f16IntegGain_Q of ' gcb ' exceeds the fixed-point range.']);
      |         end
      |         if f16IntegGain_Q<-2^15
      |           f16IntegGain_Q=-2^15;
      |           warning(['Parameter f16IntegGain_Q of ' gcb ' exceeds the fixed-point range.']);
      |         end
      |         if isnan(f16PropGain_D)
      |           if ~strcmp(f16PropGain_D_bkup,'0')
      |             set_param(gcb,'f16PropGain_D','0');
      |           end
      |         else
      |           tmps=num2str(f16PropGain_D);
      |           if ~strcmp(f16PropGain_D_bkup,tmps)
      |             set_param(gcb,'f16PropGain_D',tmps);
      |           end
      |         end
      |         if isnan(f16IntegGain_D)
      |           if ~strcmp(f16IntegGain_D_bkup,'0')
      |             set_param(gcb,'f16IntegGain_D','0');
      |           end
      |         else
      |           tmps=num2str(f16IntegGain_D);
      |           if ~strcmp(f16IntegGain_D_bkup,tmps)
      |             set_param(gcb,'f16IntegGain_D',tmps);
      |           end
      |         end
      |         if isnan(s16PropGainShift_D)
      |           if ~strcmp(s16PropGainShift_D_bkup,'0')
      |             set_param(gcb,'s16PropGainShift_D','0');
      |           end
      |         else
      |           tmps=num2str(s16PropGainShift_D);
      |           if ~strcmp(s16PropGainShift_D_bkup,tmps)
      |             set_param(gcb,'s16PropGainShift_D',tmps);
      |           end
      |         end
      |         if isnan(s16IntegGainShift_D)
      |           if ~strcmp(s16IntegGainShift_D_bkup,'0')
      |             set_param(gcb,'s16IntegGainShift_D','0');
      |           end
      |         else
      |           tmps=num2str(s16IntegGainShift_D);
      |           if ~strcmp(s16IntegGainShift_D_bkup,tmps)
      |             set_param(gcb,'s16IntegGainShift_D',tmps);
      |           end
      |         end
      |         if isnan(f16PropGain_Q)
      |           if ~strcmp(f16PropGain_Q_bkup,'0')
      |             set_param(gcb,'f16PropGain_Q','0');
      |           end
      |         else
      |           tmps=num2str(f16PropGain_Q);
      |           if ~strcmp(f16PropGain_Q_bkup,tmps)
      |             set_param(gcb,'f16PropGain_Q',tmps);
      |           end
      |         end
      |         if isnan(f16IntegGain_Q)
      |           if ~strcmp(f16IntegGain_Q_bkup,'0')
      |             set_param(gcb,'f16IntegGain_Q','0');
      |           end
      |         else
      |           tmps=num2str(f16IntegGain_Q);
      |           if ~strcmp(f16IntegGain_Q_bkup,tmps)
      |             set_param(gcb,'f16IntegGain_Q',tmps);
      |           end
      |         end
      |         if isnan(s16PropGainShift_Q)
      |           if ~strcmp(s16PropGainShift_Q_bkup,'0')
      |             set_param(gcb,'s16PropGainShift_Q','0');
      |           end
      |         else
      |           tmps=num2str(s16PropGainShift_Q);
      |           if ~strcmp(s16PropGainShift_Q_bkup,tmps)
      |             set_param(gcb,'s16PropGainShift_Q',tmps);
      |           end
      |         end
      |         if isnan(s16IntegGainShift_Q)
      |           if ~strcmp(s16IntegGainShift_Q_bkup,'0')
      |             set_param(gcb,'s16IntegGainShift_Q','0');
      |           end
      |         else
      |           tmps=num2str(s16IntegGainShift_Q);
      |           if ~strcmp(s16IntegGainShift_Q_bkup,tmps)
      |             set_param(gcb,'s16IntegGainShift_Q',tmps);
      |           end
      |         end
      |       end
      |     end
      |   catch
      |    warning(['Sample time cannot be calculated for the block ' gcb])
      |   end
      | end
      mask DialogControl timeHint Prompt: Note: Implementation parameters cannot be calculated yet because the block's inherited sample time is unknown. Simulink will update the sample time when you run the simulation.
      mask Display:
      | color('black');
      | pos = get_param(gcb, 'Position');
      | width = pos(3) - pos(1);
      | height = pos(4) - pos(2);
      | tX=width/2;
      | tY=height - 25;
      | color('black');
      | text(tX,tY, 'AMCLIB_CurrentLoopPIp_F16', 'horizontalAlignment', 'center');
      | if showStates == 2
      |   color('red');
      |   text(tX,tY - 20, ['debugging mode' char(13) char(10) '(limited performance)'], 'horizontalAlignment', 'center');
      | end
  AMCLIB_CurrentLoop_F16 : Subsystem  StartFcn=|  TreatAsAtomicUnit=on  mask(AMCLIB_CurrentLoop_F16){showStates=Hide (faster execution), resetStatesEnable=Pre-set according to the first set of inputs after reset, SampleTime=-1, intmethod=Trapezoidal, if0=350, iksi=1, Ld=3e-4, Lq=3e-4, Rs=0.33, uscale=15, iscale=10, autoCalcEn=on, f16CC1sc_D=0, f16CC2sc_D=0, u16NShift_D=0, f16CC1sc_Q=0, f16CC2sc_Q=0, u16NShift_Q=0, SampleTime_1=NaN}
      | ts=get_param(gcb,'CompiledSampleTime');
      | if iscell(ts)
      |   ts=ts{1};
      |   if iscell(ts)
      |     ts=ts{1};
      |   end
      | end
      | ts=ts(1);
      | set_param(gcb,'SampleTime_1',num2str(ts));
      | p=Simulink.Mask.get(gcb);
      | hintText=p.getDialogControl('timeHint');
      | SampleTime=Simulink.data.evalinGlobal(bdroot,get_param(gcb,'SampleTime'));
      | p=Simulink.Mask.get(gcb);
      | autoCalcEn=get_param(gcb,'autoCalcEn');
      | if strcmp(autoCalcEn,'on')
      |   if SampleTime==-1
      |     hintText.Prompt='Caution: Implementation parameters depend on inherited sample time. Make sure that the sample time of the block''s inputs corresponds to the sampling period in the target application.';
      |   else
      |     hintText.Prompt='Caution: Implementation parameters depend on the sample time. Make sure that the simulation time step corresponds to the sampling period in the target application.';
      |   end
      |   SampleTime=ts;
      |   f16CC1sc_D_bkup=get_param(gcb,'f16CC1sc_D');
      |   f16CC2sc_D_bkup=get_param(gcb,'f16CC2sc_D');
      |   u16NShift_D_bkup=get_param(gcb,'u16NShift_D');
      |   f16CC1sc_Q_bkup=get_param(gcb,'f16CC1sc_Q');
      |   f16CC2sc_Q_bkup=get_param(gcb,'f16CC2sc_Q');
      |   u16NShift_Q_bkup=get_param(gcb,'u16NShift_Q');
      |   intmethod=get_param(gcb,'intmethod');
      |   if0=Simulink.data.evalinGlobal(bdroot,get_param(gcb,'if0'));
      |   iksi=Simulink.data.evalinGlobal(bdroot,get_param(gcb,'iksi'));
      |   Ld=Simulink.data.evalinGlobal(bdroot,get_param(gcb,'Ld'));
      |   Lq=Simulink.data.evalinGlobal(bdroot,get_param(gcb,'Lq'));
      |   Rs=Simulink.data.evalinGlobal(bdroot,get_param(gcb,'Rs'));
      |   uscale=Simulink.data.evalinGlobal(bdroot,get_param(gcb,'uscale'));
      |   iscale=Simulink.data.evalinGlobal(bdroot,get_param(gcb,'iscale'));
      |   if (if0<=0)
      |     warning('Natural frequency f0 must be positive.');
      |   end
      |   if (iksi<=0)
      |     warning('Current loop attenuation must be positive.');
      |   end
      |   if (iksi>1)
      |     warning('Current loop attenuation must not exceed 1.');
      |   end
      |   if (Ld<=0)
      |     warning('Inductance Ld must be positive.');
      |   end
      |   if (Lq<=0)
      |     warning('Inductance Lq must be positive.');
      |   end
      |   if (Rs<0)
      |     warning('Resistance Rs must be non-negative.');
      |   end
      |   if (uscale<=0)
      |     warning('U_max must be positive.');
      |   end
      |   if (iscale<=0)
      |     warning('I_max must be positive.');
      |   end
      |   w0=6.283185307179586*if0;
      |   pgainD=2.0*iksi*w0*Ld-Rs;
      |   igainD=w0*w0*Ld;
      |   pgainQ=2.0*iksi*w0*Lq-Rs;
      |   igainQ=w0*w0*Lq;
      |   if strcmp(intmethod,'Forward Rectangular')
      |     cc1d=pgainD;
      |     cc2d=-pgainD+igainD*SampleTime;
      |     cc1q=pgainQ;
      |     cc2q=-pgainQ+igainQ*SampleTime;
      |   else
      |     if strcmp(intmethod,'Backward Rectangular')
      |       cc1d=pgainD+igainD*SampleTime;
      |       cc2d=-pgainD;
      |       cc1q=pgainQ+igainQ*SampleTime;
      |       cc2q=-pgainQ;
      |     else
      |       cc1d=pgainD+igainD*SampleTime*0.5;
      |       cc2d=-pgainD+igainD*SampleTime*0.5;
      |       cc1q=pgainQ+igainQ*SampleTime*0.5;
      |       cc2q=-pgainQ+igainQ*SampleTime*0.5;
      |     end
      |   end
      |   cc1fd=cc1d*iscale/uscale;
      |   cc2fd=cc2d*iscale/uscale;
      |   cc1fq=cc1q*iscale/uscale;
      |   cc2fq=cc2q*iscale/uscale;
      |   u16NShift_D=ceil(log2(abs(cc1fd)));
      |   tmpsh=ceil(log2(abs(cc2fd)));
      |   if u16NShift_D<tmpsh
      |     u16NShift_D=tmpsh;
      |   end
      |   if u16NShift_D<0
      |     u16NShift_D=0;
      |   end
      |   if u16NShift_D>15
      |     u16NShift_D=15;
      |     warning(['Parameter u16NShift_D of ' gcb ' exceeds the fixed-point range.']);
      |   end
      |   u16NShift_Q=ceil(log2(abs(cc1fq)));
      |   tmpsh=ceil(log2(abs(cc2fq)));
      |   if u16NShift_Q<tmpsh
      |     u16NShift_Q=tmpsh;
      |   end
      |   if u16NShift_Q<0
      |     u16NShift_Q=0;
      |   end
      |   if u16NShift_Q>15
      |     u16NShift_Q=15;
      |     warning(['Parameter u16NShift_Q of ' gcb ' exceeds the fixed-point range.']);
      |   end
      |   f16CC1sc_D=round(cc1fd*2^(-u16NShift_D)*2^15);
      |   if f16CC1sc_D>2^15-1
      |     f16CC1sc_D=2^15-1;
      |     warning(['Parameter f16CC1sc_D of ' gcb ' exceeds the fixed-point range.']);
      |   end
      |   if f16CC1sc_D<-2^15
      |     f16CC1sc_D=-2^15;
      |     warning(['Parameter f16CC1sc_D of ' gcb ' exceeds the fixed-point range.']);
      |   end
      |   f16CC2sc_D=round(cc2fd*2^(-u16NShift_D)*2^15);
      |   if f16CC2sc_D>2^15-1
      |     f16CC2sc_D=2^15-1;
      |     warning(['Parameter f16CC2sc_D of ' gcb ' exceeds the fixed-point range.']);
      |   end
      |   if f16CC2sc_D<-2^15
      |     f16CC2sc_D=-2^15;
      |     warning(['Parameter f16CC2sc_D of ' gcb ' exceeds the fixed-point range.']);
      |   end
      |   f16CC1sc_Q=round(cc1fq*2^(-u16NShift_Q)*2^15);
      |   if f16CC1sc_Q>2^15-1
      |     f16CC1sc_Q=2^15-1;
      |     warning(['Parameter f16CC1sc_Q of ' gcb ' exceeds the fixed-point range.']);
      |   end
      |   if f16CC1sc_Q<-2^15
      |     f16CC1sc_Q=-2^15;
      |     warning(['Parameter f16CC1sc_Q of ' gcb ' exceeds the fixed-point range.']);
      |   end
      |   f16CC2sc_Q=round(cc2fq*2^(-u16NShift_Q)*2^15);
      |   if f16CC2sc_Q>2^15-1
      |     f16CC2sc_Q=2^15-1;
      |     warning(['Parameter f16CC2sc_Q of ' gcb ' exceeds the fixed-point range.']);
      |   end
      |   if f16CC2sc_Q<-2^15
      |     f16CC2sc_Q=-2^15;
      |     warning(['Parameter f16CC2sc_Q of ' gcb ' exceeds the fixed-point range.']);
      |   end
      |   if isnan(f16CC1sc_D)
      |     if ~strcmp(f16CC1sc_D_bkup,'0')
      |       set_param(gcb,'f16CC1sc_D','0');
      |     end
      |   else
      |     tmps=num2str(f16CC1sc_D);
      |     if ~strcmp(f16CC1sc_D_bkup,tmps)
      |       set_param(gcb,'f16CC1sc_D',tmps);
      |     end
      |   end
      |   if isnan(f16CC2sc_D)
      |     if ~strcmp(f16CC2sc_D_bkup,'0')
      |       set_param(gcb,'f16CC2sc_D','0');
      |     end
      |   else
      |     tmps=num2str(f16CC2sc_D);
      |     if ~strcmp(f16CC2sc_D_bkup,tmps)
      |       set_param(gcb,'f16CC2sc_D',tmps);
      |     end
      |   end
      |   if isnan(u16NShift_D)
      |     if ~strcmp(u16NShift_D_bkup,'0')
      |       set_param(gcb,'u16NShift_D','0');
      |     end
      |   else
      |     tmps=num2str(u16NShift_D);
      |     if ~strcmp(u16NShift_D_bkup,tmps)
      |       set_param(gcb,'u16NShift_D',tmps);
      |     end
      |   end
      |   if isnan(f16CC1sc_Q)
      |     if ~strcmp(f16CC1sc_Q_bkup,'0')
      |       set_param(gcb,'f16CC1sc_Q','0');
      |     end
      |   else
      |     tmps=num2str(f16CC1sc_Q);
      |     if ~strcmp(f16CC1sc_Q_bkup,tmps)
      |       set_param(gcb,'f16CC1sc_Q',tmps);
      |     end
      |   end
      |   if isnan(f16CC2sc_Q)
      |     if ~strcmp(f16CC2sc_Q_bkup,'0')
      |       set_param(gcb,'f16CC2sc_Q','0');
      |     end
      |   else
      |     tmps=num2str(f16CC2sc_Q);
      |     if ~strcmp(f16CC2sc_Q_bkup,tmps)
      |       set_param(gcb,'f16CC2sc_Q',tmps);
      |     end
      |   end
      |   if isnan(u16NShift_Q)
      |     if ~strcmp(u16NShift_Q_bkup,'0')
      |       set_param(gcb,'u16NShift_Q','0');
      |     end
      |   else
      |     tmps=num2str(u16NShift_Q);
      |     if ~strcmp(u16NShift_Q_bkup,tmps)
      |       set_param(gcb,'u16NShift_Q',tmps);
      |     end
      |   end
      | end
      mask prompts: showStates "Show internal states:"; resetStatesEnable "Internal state after reset:"; SampleTime "Sample time (-1 for inherited):"; intmethod "Integration method:"; if0 "Current loop natural frequency f0 [Hz]:"; iksi "Current loop attenuation ξ:"; Ld "D-axis stator inductance Ld [H]"; Lq "Q-axis stator inductance Lq [H]"; Rs "Winding resistance Rs [ohm]:"; uscale "U_max (maximum DC bus voltage) [V]:"; iscale "I_max (maximum phase current) [A]:"; autoCalcEn "Calculate implementation parameters from physical parameters"; f16CC1sc_D "f16CC1sc_D (CC1 coefficient of the D-axis PI controller):"; f16CC2sc_D "f16CC2sc_D (CC2 coefficient of the D-axis PI controller):"; u16NShift_D "u16NShift_D (Scaling bitwise shift applied to the D-axis controller coefficients):"; f16CC1sc_Q "f16CC1sc_Q (CC1 coefficient of the Q-axis PI controller):"; f16CC2sc_Q "f16CC2sc_Q (CC2 coefficient of the Q-axis PI controller):"; u16NShift_Q "u16NShift_Q (Scaling bitwise shift applied to the Q-axis controller coefficients):"; SampleTime_1 "Discrete sample time:"
      mask help: Current control loop of the PMSM field-oriented control algorithm in 16-bit fixed-point fractional implementation. The current control loop contains two PI controllers in recurrent form. This block supports re-initialization of the internal state during simulation. If the block is reset, the outputs of the PI controllers will be aligned with the inputs f16ControllerPIrAWDOut_preset and f16ControllerPIrAWQOut_preset. Refer to the AMMCLIB User's Guide for further details.
      mask init:
      | ddName = get_param(bdroot,'DataDictionary');
      | if length(ddName)==0
      |   set_param(bdroot,'DataDictionary','ammclib_types.sldd');
      | else
      |   dd = Simulink.data.dictionary.open(ddName);
      |   data = getSection(dd,'Design Data');
      |   if ~exist(data,'SWLIBS_2Syst_F16')
      |     addDataSource(dd,'ammclib_types.sldd');
      |     saveChanges(dd);
      |   end
      | end
      | 
      | if showStates == 1
      |   % hidden state variables
      |   if strcmp(get_param([gcb '/f16CC1sc_D'], 'BlockType'), 'Inport')
      |     posblk = get_param(gcb, 'Position');
      | 
      |     pos = get_param([gcb, '/f16CC1sc_D'], 'Position');
      |     orient = get_param([gcb, '/f16CC1sc_D'], 'Orientation');
      |     delete_block([gcb, '/f16CC1sc_D']);
      |     add_block('built-in/Ground', [gcb, '/f16CC1sc_D'], 'Position', pos, 'Orientation', orient);
      | 
      |     pos = get_param([gcb, '/f16CC2sc_D'], 'Position');
      |     orient = get_param([gcb, '/f16CC2sc_D'], 'Orientation');
      |     delete_block([gcb, '/f16CC2sc_D']);
      |     add_block('built-in/Ground', [gcb, '/f16CC2sc_D'], 'Position', pos, 'Orientation', orient);
      | 
      |     pos = get_param([gcb, '/u16NShift_D'], 'Position');
      |     orient = get_param([gcb, '/u16NShift_D'], 'Orientation');
      |     delete_block([gcb, '/u16NShift_D']);
      |     add_block('built-in/Ground', [gcb, '/u16NShift_D'], 'Position', pos, 'Orientation', orient);
      | 
      |     pos = get_param([gcb, '/f16CC1sc_Q'], 'Position');
      |     orient = get_param([gcb, '/f16CC1sc_Q'], 'Orientation');
      |     delete_block([gcb, '/f16CC1sc_Q']);
      |     add_block('built-in/Ground', [gcb, '/f16CC1sc_Q'], 'Position', pos, 'Orientation', orient);
      | 
      |     pos = get_param([gcb, '/f16CC2sc_Q'], 'Position');
      |     orient = get_param([gcb, '/f16CC2sc_Q'], 'Orientation');
      |     delete_block([gcb, '/f16CC2sc_Q']);
      |     add_block('built-in/Ground', [gcb, '/f16CC2sc_Q'], 'Position', pos, 'Orientation', orient);
      | 
      |     pos = get_param([gcb, '/u16NShift_Q'], 'Position');
      |     orient = get_param([gcb, '/u16NShift_Q'], 'Orientation');
      |     delete_block([gcb, '/u16NShift_Q']);
      |     add_block('built-in/Ground', [gcb, '/u16NShift_Q'], 'Position', pos, 'Orientation', orient);
      | 
      |     pos = get_param([gcb, '/f32Acc_D'], 'Position');
      |     orient = get_param([gcb, '/f32Acc_D'], 'Orientation');
      |     delete_block([gcb, '/f32Acc_D']);
      |     add_block('built-in/Ground', [gcb, '/f32Acc_D'], 'Position', pos, 'Orientation', orient);
      | 
      |     pos = get_param([gcb, '/f16InErrK1_D'], 'Position');
      |     orient = get_param([gcb, '/f16InErrK1_D'], 'Orientation');
      |     delete_block([gcb, '/f16InErrK1_D']);
      |     add_block('built-in/Ground', [gcb, '/f16InErrK1_D'], 'Position', pos, 'Orientation', orient);
      | 
      |     pos = get_param([gcb, '/f32Acc_Q'], 'Position');
      |     orient = get_param([gcb, '/f32Acc_Q'], 'Orientation');
      |     delete_block([gcb, '/f32Acc_Q']);
      |     add_block('built-in/Ground', [gcb, '/f32Acc_Q'], 'Position', pos, 'Orientation', orient);
      | 
      |     pos = get_param([gcb, '/f16InErrK1_Q'], 'Position');
      |     orient = get_param([gcb, '/f16InErrK1_Q'], 'Orientation');
      |     delete_block([gcb, '/f16InErrK1_Q']);
      |     add_block('built-in/Ground', [gcb, '/f16InErrK1_Q'], 'Position', pos, 'Orientation', orient);
      | 
      | 
      |     pmask=Simulink.Mask.get(gcb);
      |     pctrl=pmask.getParameter('SampleTime');
      |     pctrl.set('TypeOptions',{'f16UDcBus/SampleTime','pIDQReq/SampleTime','pIDQFbck/SampleTime','f16ControllerPIrAWDOut_preset/SampleTime','f16ControllerPIrAWQOut_preset/SampleTime'});
      | 
      |     pos = get_param([gcb '/f32Acc_D_Out'], 'Position');
      |     orient = get_param([gcb '/f32Acc_D_Out'], 'Orientation');
      |     delete_block([gcb '/f32Acc_D_Out']);
      |     add_block('built-in/Terminator', [gcb '/f32Acc_D_Out'], 'Position', pos, 'Orientation', orient);
      | 
      |     pos = get_param([gcb '/f16InErrK1_D_Out'], 'Position');
      |     orient = get_param([gcb '/f16InErrK1_D_Out'], 'Orientation');
      |     delete_block([gcb '/f16InErrK1_D_Out']);
      |     add_block('built-in/Terminator', [gcb '/f16InErrK1_D_Out'], 'Position', pos, 'Orientation', orient);
      | 
      |     pos = get_param([gcb '/f32Acc_Q_Out'], 'Position');
      |     orient = get_param([gcb '/f32Acc_Q_Out'], 'Orientation');
      |     delete_block([gcb '/f32Acc_Q_Out']);
      |     add_block('built-in/Terminator', [gcb '/f32Acc_Q_Out'], 'Position', pos, 'Orientation', orient);
      | 
      |     pos = get_param([gcb '/f16InErrK1_Q_Out'], 'Position');
      |     orient = get_param([gcb '/f16InErrK1_Q_Out'], 'Orientation');
      |     delete_block([gcb '/f16InErrK1_Q_Out']);
      |     add_block('built-in/Terminator', [gcb '/f16InErrK1_Q_Out'], 'Position', pos, 'Orientation', orient);
      | 
      |     set_param([gcb '/f16UDcBus'], 'Port', '1');
      |     set_param([gcb '/pIDQReq'], 'Port', '2');
      |     set_param([gcb '/pIDQFbck'], 'Port', '3');
      |     set_param([gcb '/f16ControllerPIrAWDOut_preset'], 'Port', '4');
      |     set_param([gcb '/f16ControllerPIrAWQOut_preset'], 'Port', '5');
      | 
      |     tmpOutCnt=0;
      |     tmpOutCnt=tmpOutCnt+1;
      |     set_param([gcb '/pUDQReq'], 'Port', num2str(tmpOutCnt));
      |     tmpOutCnt=tmpOutCnt+1;
      |     set_param([gcb '/f16UQLim'], 'Port', num2str(tmpOutCnt));
      | 
      |     autoCalcEn=get_param(gcb,'autoCalcEn');
      |     if strcmp(autoCalcEn,'on')
      |       set_param(gcb,'MaskEnables',{'on','on','on','on','on','on','on','on','on','on','on','on','on','on','on','on','on','on','off'});
      |     else
      |       set_param(gcb,'MaskEnables',{'on','on','on','off','off','off','off','off','off','off','off','on','on','on','on','on','on','on','off'});
      |     end
      | 
      |     if (posblk(4) - posblk(2)) > 150
      |       height = 150;
      |       set_param(gcb,'Position',[posblk(1), posblk(2), posblk(3), posblk(2)+height])
      |     end
      |   end
      | else
      |   % shown state variables
      |   if strcmp(get_param([gcb '/f16CC1sc_D'], 'BlockType'), 'Ground')
      |     posblk = get_param(gcb, 'Position');
      | 
      |     pos = get_param([gcb, '/f16CC1sc_D'], 'Position');
      |     orient = get_param([gcb, '/f16CC1sc_D'], 'Orientation');
      |     delete_block([gcb, '/f16CC1sc_D']);
      |     add_block('built-in/Inport', [gcb, '/f16CC1sc_D'], 'Position', pos, 'Orientation', orient, 'OutDataTypeStr', 'int16');
      | 
      |     pos = get_param([gcb, '/f16CC2sc_D'], 'Position');
      |     orient = get_param([gcb, '/f16CC2sc_D'], 'Orientation');
      |     delete_block([gcb, '/f16CC2sc_D']);
      |     add_block('built-in/Inport', [gcb, '/f16CC2sc_D'], 'Position', pos, 'Orientation', orient, 'OutDataTypeStr', 'int16');
      | 
      |     pos = get_param([gcb, '/u16NShift_D'], 'Position');
      |     orient = get_param([gcb, '/u16NShift_D'], 'Orientation');
      |     delete_block([gcb, '/u16NShift_D']);
      |     add_block('built-in/Inport', [gcb, '/u16NShift_D'], 'Position', pos, 'Orientation', orient, 'OutDataTypeStr', 'uint16');
      | 
      |     pos = get_param([gcb, '/f16CC1sc_Q'], 'Position');
      |     orient = get_param([gcb, '/f16CC1sc_Q'], 'Orientation');
      |     delete_block([gcb, '/f16CC1sc_Q']);
      |     add_block('built-in/Inport', [gcb, '/f16CC1sc_Q'], 'Position', pos, 'Orientation', orient, 'OutDataTypeStr', 'int16');
      | 
      |     pos = get_param([gcb, '/f16CC2sc_Q'], 'Position');
      |     orient = get_param([gcb, '/f16CC2sc_Q'], 'Orientation');
      |     delete_block([gcb, '/f16CC2sc_Q']);
      |     add_block('built-in/Inport', [gcb, '/f16CC2sc_Q'], 'Position', pos, 'Orientation', orient, 'OutDataTypeStr', 'int16');
      | 
      |     pos = get_param([gcb, '/u16NShift_Q'], 'Position');
      |     orient = get_param([gcb, '/u16NShift_Q'], 'Orientation');
      |     delete_block([gcb, '/u16NShift_Q']);
      |     add_block('built-in/Inport', [gcb, '/u16NShift_Q'], 'Position', pos, 'Orientation', orient, 'OutDataTypeStr', 'uint16');
      | 
      |     pos = get_param([gcb, '/f32Acc_D'], 'Position');
      |     orient = get_param([gcb, '/f32Acc_D'], 'Orientation');
      |     delete_block([gcb, '/f32Acc_D']);
      |     add_block('built-in/Inport', [gcb, '/f32Acc_D'], 'Position', pos, 'Orientation', orient, 'OutDataTypeStr', 'int32');
      | 
      |     pos = get_param([gcb, '/f16InErrK1_D'], 'Position');
      |     orient = get_param([gcb, '/f16InErrK1_D'], 'Orientation');
      |     delete_block([gcb, '/f16InErrK1_D']);
      |     add_block('built-in/Inport', [gcb, '/f16InErrK1_D'], 'Position', pos, 'Orientation', orient, 'OutDataTypeStr', 'int16');
      | 
      |     pos = get_param([gcb, '/f32Acc_Q'], 'Position');
      |     orient = get_param([gcb, '/f32Acc_Q'], 'Orientation');
      |     delete_block([gcb, '/f32Acc_Q']);
      |     add_block('built-in/Inport', [gcb, '/f32Acc_Q'], 'Position', pos, 'Orientation', orient, 'OutDataTypeStr', 'int32');
      | 
      |     pos = get_param([gcb, '/f16InErrK1_Q'], 'Position');
      |     orient = get_param([gcb, '/f16InErrK1_Q'], 'Orientation');
      |     delete_block([gcb, '/f16InErrK1_Q']);
      |     add_block('built-in/Inport', [gcb, '/f16InErrK1_Q'], 'Position', pos, 'Orientation', orient, 'OutDataTypeStr', 'int16');
      | 
      | 
      | 
      |     pos = get_param([gcb '/f32Acc_D_Out'], 'Position');
      |     orient = get_param([gcb '/f32Acc_D_Out'], 'Orientation');
      |     delete_block([gcb '/f32Acc_D_Out']);
      |     add_block('built-in/Outport', [gcb '/f32Acc_D_Out'], 'Position', pos, 'Orientation', orient);
      | 
      |     pos = get_param([gcb '/f16InErrK1_D_Out'], 'Position');
      |     orient = get_param([gcb '/f16InErrK1_D_Out'], 'Orientation');
      |     delete_block([gcb '/f16InErrK1_D_Out']);
      |     add_block('built-in/Outport', [gcb '/f16InErrK1_D_Out'], 'Position', pos, 'Orientation', orient);
      | 
      |     pos = get_param([gcb '/f32Acc_Q_Out'], 'Position');
      |     orient = get_param([gcb '/f32Acc_Q_Out'], 'Orientation');
      |     delete_block([gcb '/f32Acc_Q_Out']);
      |     add_block('built-in/Outport', [gcb '/f32Acc_Q_Out'], 'Position', pos, 'Orientation', orient);
      | 
      |     pos = get_param([gcb '/f16InErrK1_Q_Out'], 'Position');
      |     orient = get_param([gcb '/f16InErrK1_Q_Out'], 'Orientation');
      |     delete_block([gcb '/f16InErrK1_Q_Out']);
      |     add_block('built-in/Outport', [gcb '/f16InErrK1_Q_Out'], 'Position', pos, 'Orientation', orient);
      | 
      | 
      |     pmask=Simulink.Mask.get(gcb);
      |     pctrl=pmask.getParameter('SampleTime');
      |     pctrl.set('TypeOptions',{'f16UDcBus/SampleTime','pIDQReq/SampleTime','pIDQFbck/SampleTime','f16ControllerPIrAWDOut_preset/SampleTime','f16ControllerPIrAWQOut_preset/SampleTime','f16CC1sc_D/SampleTime','f16CC2sc_D/SampleTime','u16NShift_D/SampleTime','f16CC1sc_Q/SampleTime','f16CC2sc_Q/SampleTime','u16NShift_Q/SampleTime','f32Acc_D/SampleTime','f16InErrK1_D/SampleTime','f32Acc_Q/SampleTime','f16InErrK1_Q/SampleTime'});
      | 
      |     set_param([gcb '/f16UDcBus'], 'Port', '1');
      |     set_param([gcb '/pIDQReq'], 'Port', '2');
      |     set_param([gcb '/pIDQFbck'], 'Port', '3');
      |     set_param([gcb '/f16ControllerPIrAWDOut_preset'], 'Port', '4');
      |     set_param([gcb '/f16ControllerPIrAWQOut_preset'], 'Port', '5');
      |     set_param([gcb '/f16CC1sc_D'], 'Port', '6');
      |     set_param([gcb '/f16CC2sc_D'], 'Port', '7');
      |     set_param([gcb '/u16NShift_D'], 'Port', '8');
      |     set_param([gcb '/f16CC1sc_Q'], 'Port', '9');
      |     set_param([gcb '/f16CC2sc_Q'], 'Port', '10');
      |     set_param([gcb '/u16NShift_Q'], 'Port', '11');
      |     set_param([gcb '/f32Acc_D'], 'Port', '12');
      |     set_param([gcb '/f16InErrK1_D'], 'Port', '13');
      |     set_param([gcb '/f32Acc_Q'], 'Port', '14');
      |     set_param([gcb '/f16InErrK1_Q'], 'Port', '15');
      | 
      |     tmpOutCnt=0;
      |     tmpOutCnt=tmpOutCnt+1;
      |     set_param([gcb '/pUDQReq'], 'Port', num2str(tmpOutCnt));
      |     tmpOutCnt=tmpOutCnt+1;
      |     set_param([gcb '/f16UQLim'], 'Port', num2str(tmpOutCnt));
      |     tmpOutCnt=tmpOutCnt+1;
      |     set_param([gcb '/f32Acc_D_Out'], 'Port', num2str(tmpOutCnt));
      |     tmpOutCnt=tmpOutCnt+1;
      |     set_param([gcb '/f16InErrK1_D_Out'], 'Port', num2str(tmpOutCnt));
      |     tmpOutCnt=tmpOutCnt+1;
      |     set_param([gcb '/f32Acc_Q_Out'], 'Port', num2str(tmpOutCnt));
      |     tmpOutCnt=tmpOutCnt+1;
      |     set_param([gcb '/f16InErrK1_Q_Out'], 'Port', num2str(tmpOutCnt));
      | 
      |     set_param(gcb,'MaskEnables',{'on','on','on','off','off','off','off','off','off','off','off','off','off','off','off','off','off','off','off'});
      | 
      |     if (posblk(4) - posblk(2)) < 400
      |       height = 400;
      |       set_param(gcb,'Position',[posblk(1), posblk(2), posblk(3), posblk(2)+height])
      |     end
      |   end
      | end
      settings: RTWSystemCode=Inline
      mask Help: web([fileparts(which('ammclib_bam_S32K3xx.slx')) '/../doc/S32K3XXMCLUG.pdf'], '-browser')
      mask TypeOptions showStates: Hide (faster execution) | Show (allows debugging; connect feedback loops manually)
      mask Callback showStates:
      | maskStr=get_param(gcb,'showStates');
      | if strcmp(maskStr,'Hide (faster execution)')
      |   if strcmp(get_param([gcb '/f16CC1sc_D'], 'BlockType'), 'Inport')
      |     autoCalcEn=get_param(gcb,'autoCalcEn');
      |     if strcmp(autoCalcEn,'on')
      |       set_param(gcb,'MaskEnables',{'on','on','on','on','on','on','on','on','on','on','on','on','on','on','on','on','on','on','off'});
      |     else
      |       set_param(gcb,'MaskEnables',{'on','on','on','off','off','off','off','off','off','off','off','on','on','on','on','on','on','on','off'});
      |     end
      |   end
      | else
      |   if strcmp(get_param([gcb '/f16CC1sc_D'], 'BlockType'), 'Ground')
      |     set_param(gcb,'MaskEnables',{'on','on','on','off','off','off','off','off','off','off','off','off','off','off','off','off','off','off','off'});
      |   end
      | end
      mask TypeOptions resetStatesEnable: Pre-set according to the first set of inputs after reset | Clear to zero
      mask TypeOptions SampleTime: f16UDcBus/SampleTime | pIDQReq/SampleTime | pIDQFbck/SampleTime | f16ControllerPIrAWDOut_preset/SampleTime | f16ControllerPIrAWQOut_preset/SampleTime
      mask Callback SampleTime:
      | p=Simulink.Mask.get(gcb);
      | hintText=p.getDialogControl('timeHint');
      | SampleTime=Simulink.data.evalinGlobal(bdroot,get_param(gcb,'SampleTime'));
      | SampleTime_1=str2double(get_param(gcb,'SampleTime_1'));
      | if (((SampleTime==-1) && (~contains(hintText.Prompt,'inherited'))) || ...
      |     ((SampleTime~=-1) && contains(hintText.Prompt,'inherited')) || ...
      |     ((SampleTime~=-1) && (SampleTime_1~=SampleTime)) || ...
      |     ((SampleTime_1~=-1) && contains(hintText.Prompt,'yet')))
      |   if ((SampleTime==-1) && (~contains(hintText.Prompt,'inherited')))
      |     set_param(gcb,'SampleTime_1',num2str(NaN));
      |     SampleTime_1=NaN;
      |   end
      |   if (SampleTime~=-1)
      |     set_param(gcb,'SampleTime_1',num2str(SampleTime));
      |     SampleTime_1=SampleTime;
      |   end
      |   autoCalcEn=get_param(gcb,'autoCalcEn');
      |   if strcmp(autoCalcEn,'on')
      |     p=Simulink.Mask.get(gcb);
      |     hintText=p.getDialogControl('timeHint');
      |     if SampleTime==-1
      |       SampleTime=SampleTime_1;
      |       if isnan(SampleTime)
      |         hintText.Prompt='Note: Implementation parameters cannot be calculated yet because the block''s inherited sample time is unknown. Simulink will update the sample time when you run the simulation.';
      |       else
      |         hintText.Prompt='Caution: Implementation parameters depend on inherited sample time. Make sure that the sample time of the block''s inputs corresponds to the sampling period in the target application.';
      |       end
      |     else
      |       hintText.Prompt='Caution: Implementation parameters depend on the sample time. Make sure that the simulation time step corresponds to the sampling period in the target application.';
      |     end
      |     f16CC1sc_D_bkup=get_param(gcb,'f16CC1sc_D');
      |     f16CC2sc_D_bkup=get_param(gcb,'f16CC2sc_D');
      |     u16NShift_D_bkup=get_param(gcb,'u16NShift_D');
      |     f16CC1sc_Q_bkup=get_param(gcb,'f16CC1sc_Q');
      |     f16CC2sc_Q_bkup=get_param(gcb,'f16CC2sc_Q');
      |     u16NShift_Q_bkup=get_param(gcb,'u16NShift_Q');
      |     intmethod=get_param(gcb,'intmethod');
      |     if0=Simulink.data.evalinGlobal(bdroot,get_param(gcb,'if0'));
      |     iksi=Simulink.data.evalinGlobal(bdroot,get_param(gcb,'iksi'));
      |     Ld=Simulink.data.evalinGlobal(bdroot,get_param(gcb,'Ld'));
      |     Lq=Simulink.data.evalinGlobal(bdroot,get_param(gcb,'Lq'));
      |     Rs=Simulink.data.evalinGlobal(bdroot,get_param(gcb,'Rs'));
      |     uscale=Simulink.data.evalinGlobal(bdroot,get_param(gcb,'uscale'));
      |     iscale=Simulink.data.evalinGlobal(bdroot,get_param(gcb,'iscale'));
      |     if (if0<=0)
      |       warning('Natural frequency f0 must be positive.');
      |     end
      |     if (iksi<=0)
      |       warning('Current loop attenuation must be positive.');
      |     end
      |     if (iksi>1)
      |       warning('Current loop attenuation must not exceed 1.');
      |     end
      |     if (Ld<=0)
      |       warning('Inductance Ld must be positive.');
      |     end
      |     if (Lq<=0)
      |       warning('Inductance Lq must be positive.');
      |     end
      |     if (Rs<0)
      |       warning('Resistance Rs must be non-negative.');
      |     end
      |     if (uscale<=0)
      |       warning('U_max must be positive.');
      |     end
      |     if (iscale<=0)
      |       warning('I_max must be positive.');
      |     end
      |     w0=6.283185307179586*if0;
      |     pgainD=2.0*iksi*w0*Ld-Rs;
      |     igainD=w0*w0*Ld;
      |     pgainQ=2.0*iksi*w0*Lq-Rs;
      |     igainQ=w0*w0*Lq;
      |     if strcmp(intmethod,'Forward Rectangular')
      |       cc1d=pgainD;
      |       cc2d=-pgainD+igainD*SampleTime;
      |       cc1q=pgainQ;
      |       cc2q=-pgainQ+igainQ*SampleTime;
      |     else
      |       if strcmp(intmethod,'Backward Rectangular')
      |         cc1d=pgainD+igainD*SampleTime;
      |         cc2d=-pgainD;
      |         cc1q=pgainQ+igainQ*SampleTime;
      |         cc2q=-pgainQ;
      |       else
      |         cc1d=pgainD+igainD*SampleTime*0.5;
      |         cc2d=-pgainD+igainD*SampleTime*0.5;
      |         cc1q=pgainQ+igainQ*SampleTime*0.5;
      |         cc2q=-pgainQ+igainQ*SampleTime*0.5;
      |       end
      |     end
      |     cc1fd=cc1d*iscale/uscale;
      |     cc2fd=cc2d*iscale/uscale;
      |     cc1fq=cc1q*iscale/uscale;
      |     cc2fq=cc2q*iscale/uscale;
      |     u16NShift_D=ceil(log2(abs(cc1fd)));
      |     tmpsh=ceil(log2(abs(cc2fd)));
      |     if u16NShift_D<tmpsh
      |       u16NShift_D=tmpsh;
      |     end
      |     if u16NShift_D<0
      |       u16NShift_D=0;
      |     end
      |     if u16NShift_D>15
      |       u16NShift_D=15;
      |       warning(['Parameter u16NShift_D of ' gcb ' exceeds the fixed-point range.']);
      |     end
      |     u16NShift_Q=ceil(log2(abs(cc1fq)));
      |     tmpsh=ceil(log2(abs(cc2fq)));
      |     if u16NShift_Q<tmpsh
      |       u16NShift_Q=tmpsh;
      |     end
      |     if u16NShift_Q<0
      |       u16NShift_Q=0;
      |     end
      |     if u16NShift_Q>15
      |       u16NShift_Q=15;
      |       warning(['Parameter u16NShift_Q of ' gcb ' exceeds the fixed-point range.']);
      |     end
      |     f16CC1sc_D=round(cc1fd*2^(-u16NShift_D)*2^15);
      |     if f16CC1sc_D>2^15-1
      |       f16CC1sc_D=2^15-1;
      |       warning(['Parameter f16CC1sc_D of ' gcb ' exceeds the fixed-point range.']);
      |     end
      |     if f16CC1sc_D<-2^15
      |       f16CC1sc_D=-2^15;
      |       warning(['Parameter f16CC1sc_D of ' gcb ' exceeds the fixed-point range.']);
      |     end
      |     f16CC2sc_D=round(cc2fd*2^(-u16NShift_D)*2^15);
      |     if f16CC2sc_D>2^15-1
      |       f16CC2sc_D=2^15-1;
      |       warning(['Parameter f16CC2sc_D of ' gcb ' exceeds the fixed-point range.']);
      |     end
      |     if f16CC2sc_D<-2^15
      |       f16CC2sc_D=-2^15;
      |       warning(['Parameter f16CC2sc_D of ' gcb ' exceeds the fixed-point range.']);
      |     end
      |     f16CC1sc_Q=round(cc1fq*2^(-u16NShift_Q)*2^15);
      |     if f16CC1sc_Q>2^15-1
      |       f16CC1sc_Q=2^15-1;
      |       warning(['Parameter f16CC1sc_Q of ' gcb ' exceeds the fixed-point range.']);
      |     end
      |     if f16CC1sc_Q<-2^15
      |       f16CC1sc_Q=-2^15;
      |       warning(['Parameter f16CC1sc_Q of ' gcb ' exceeds the fixed-point range.']);
      |     end
      |     f16CC2sc_Q=round(cc2fq*2^(-u16NShift_Q)*2^15);
      |     if f16CC2sc_Q>2^15-1
      |       f16CC2sc_Q=2^15-1;
      |       warning(['Parameter f16CC2sc_Q of ' gcb ' exceeds the fixed-point range.']);
      |     end
      |     if f16CC2sc_Q<-2^15
      |       f16CC2sc_Q=-2^15;
      |       warning(['Parameter f16CC2sc_Q of ' gcb ' exceeds the fixed-point range.']);
      |     end
      |     if isnan(f16CC1sc_D)
      |       if ~strcmp(f16CC1sc_D_bkup,'0')
      |         set_param(gcb,'f16CC1sc_D','0');
      |       end
      |     else
      |       tmps=num2str(f16CC1sc_D);
      |       if ~strcmp(f16CC1sc_D_bkup,tmps)
      |         set_param(gcb,'f16CC1sc_D',tmps);
      |       end
      |     end
      |     if isnan(f16CC2sc_D)
      |       if ~strcmp(f16CC2sc_D_bkup,'0')
      |         set_param(gcb,'f16CC2sc_D','0');
      |       end
      |     else
      |       tmps=num2str(f16CC2sc_D);
      |       if ~strcmp(f16CC2sc_D_bkup,tmps)
      |         set_param(gcb,'f16CC2sc_D',tmps);
      |       end
      |     end
      |     if isnan(u16NShift_D)
      |       if ~strcmp(u16NShift_D_bkup,'0')
      |         set_param(gcb,'u16NShift_D','0');
      |       end
      |     else
      |       tmps=num2str(u16NShift_D);
      |       if ~strcmp(u16NShift_D_bkup,tmps)
      |         set_param(gcb,'u16NShift_D',tmps);
      |       end
      |     end
      |     if isnan(f16CC1sc_Q)
      |       if ~strcmp(f16CC1sc_Q_bkup,'0')
      |         set_param(gcb,'f16CC1sc_Q','0');
      |       end
      |     else
      |       tmps=num2str(f16CC1sc_Q);
      |       if ~strcmp(f16CC1sc_Q_bkup,tmps)
      |         set_param(gcb,'f16CC1sc_Q',tmps);
      |       end
      |     end
      |     if isnan(f16CC2sc_Q)
      |       if ~strcmp(f16CC2sc_Q_bkup,'0')
      |         set_param(gcb,'f16CC2sc_Q','0');
      |       end
      |     else
      |       tmps=num2str(f16CC2sc_Q);
      |       if ~strcmp(f16CC2sc_Q_bkup,tmps)
      |         set_param(gcb,'f16CC2sc_Q',tmps);
      |       end
      |     end
      |     if isnan(u16NShift_Q)
      |       if ~strcmp(u16NShift_Q_bkup,'0')
      |         set_param(gcb,'u16NShift_Q','0');
      |       end
      |     else
      |       tmps=num2str(u16NShift_Q);
      |       if ~strcmp(u16NShift_Q_bkup,tmps)
      |         set_param(gcb,'u16NShift_Q',tmps);
      |       end
      |     end
      |   end
      | end
      mask TypeOptions intmethod: Forward Rectangular | Backward Rectangular | Trapezoidal
      mask Callback intmethod:
      | autoCalcEn=get_param(gcb,'autoCalcEn');
      | if strcmp(autoCalcEn,'on')
      |   SampleTime=Simulink.data.evalinGlobal(bdroot,get_param(gcb,'SampleTime'));
      |   if (SampleTime==-1)
      |     SampleTime=str2double(get_param(gcb,'SampleTime_1'));
      |   end
      |   f16CC1sc_D_bkup=get_param(gcb,'f16CC1sc_D');
      |   f16CC2sc_D_bkup=get_param(gcb,'f16CC2sc_D');
      |   u16NShift_D_bkup=get_param(gcb,'u16NShift_D');
      |   f16CC1sc_Q_bkup=get_param(gcb,'f16CC1sc_Q');
      |   f16CC2sc_Q_bkup=get_param(gcb,'f16CC2sc_Q');
      |   u16NShift_Q_bkup=get_param(gcb,'u16NShift_Q');
      |   intmethod=get_param(gcb,'intmethod');
      |   if0=Simulink.data.evalinGlobal(bdroot,get_param(gcb,'if0'));
      |   iksi=Simulink.data.evalinGlobal(bdroot,get_param(gcb,'iksi'));
      |   Ld=Simulink.data.evalinGlobal(bdroot,get_param(gcb,'Ld'));
      |   Lq=Simulink.data.evalinGlobal(bdroot,get_param(gcb,'Lq'));
      |   Rs=Simulink.data.evalinGlobal(bdroot,get_param(gcb,'Rs'));
      |   uscale=Simulink.data.evalinGlobal(bdroot,get_param(gcb,'uscale'));
      |   iscale=Simulink.data.evalinGlobal(bdroot,get_param(gcb,'iscale'));
      |   if (if0<=0)
      |     warning('Natural frequency f0 must be positive.');
      |   end
      |   if (iksi<=0)
      |     warning('Current loop attenuation must be positive.');
      |   end
      |   if (iksi>1)
      |     warning('Current loop attenuation must not exceed 1.');
      |   end
      |   if (Ld<=0)
      |     warning('Inductance Ld must be positive.');
      |   end
      |   if (Lq<=0)
      |     warning('Inductance Lq must be positive.');
      |   end
      |   if (Rs<0)
      |     warning('Resistance Rs must be non-negative.');
      |   end
      |   if (uscale<=0)
      |     warning('U_max must be positive.');
      |   end
      |   if (iscale<=0)
      |     warning('I_max must be positive.');
      |   end
      |   w0=6.283185307179586*if0;
      |   pgainD=2.0*iksi*w0*Ld-Rs;
      |   igainD=w0*w0*Ld;
      |   pgainQ=2.0*iksi*w0*Lq-Rs;
      |   igainQ=w0*w0*Lq;
      |   if strcmp(intmethod,'Forward Rectangular')
      |     cc1d=pgainD;
      |     cc2d=-pgainD+igainD*SampleTime;
      |     cc1q=pgainQ;
      |     cc2q=-pgainQ+igainQ*SampleTime;
      |   else
      |     if strcmp(intmethod,'Backward Rectangular')
      |       cc1d=pgainD+igainD*SampleTime;
      |       cc2d=-pgainD;
      |       cc1q=pgainQ+igainQ*SampleTime;
      |       cc2q=-pgainQ;
      |     else
      |       cc1d=pgainD+igainD*SampleTime*0.5;
      |       cc2d=-pgainD+igainD*SampleTime*0.5;
      |       cc1q=pgainQ+igainQ*SampleTime*0.5;
      |       cc2q=-pgainQ+igainQ*SampleTime*0.5;
      |     end
      |   end
      |   cc1fd=cc1d*iscale/uscale;
      |   cc2fd=cc2d*iscale/uscale;
      |   cc1fq=cc1q*iscale/uscale;
      |   cc2fq=cc2q*iscale/uscale;
      |   u16NShift_D=ceil(log2(abs(cc1fd)));
      |   tmpsh=ceil(log2(abs(cc2fd)));
      |   if u16NShift_D<tmpsh
      |     u16NShift_D=tmpsh;
      |   end
      |   if u16NShift_D<0
      |     u16NShift_D=0;
      |   end
      |   if u16NShift_D>15
      |     u16NShift_D=15;
      |     warning(['Parameter u16NShift_D of ' gcb ' exceeds the fixed-point range.']);
      |   end
      |   u16NShift_Q=ceil(log2(abs(cc1fq)));
      |   tmpsh=ceil(log2(abs(cc2fq)));
      |   if u16NShift_Q<tmpsh
      |     u16NShift_Q=tmpsh;
      |   end
      |   if u16NShift_Q<0
      |     u16NShift_Q=0;
      |   end
      |   if u16NShift_Q>15
      |     u16NShift_Q=15;
      |     warning(['Parameter u16NShift_Q of ' gcb ' exceeds the fixed-point range.']);
      |   end
      |   f16CC1sc_D=round(cc1fd*2^(-u16NShift_D)*2^15);
      |   if f16CC1sc_D>2^15-1
      |     f16CC1sc_D=2^15-1;
      |     warning(['Parameter f16CC1sc_D of ' gcb ' exceeds the fixed-point range.']);
      |   end
      |   if f16CC1sc_D<-2^15
      |     f16CC1sc_D=-2^15;
      |     warning(['Parameter f16CC1sc_D of ' gcb ' exceeds the fixed-point range.']);
      |   end
      |   f16CC2sc_D=round(cc2fd*2^(-u16NShift_D)*2^15);
      |   if f16CC2sc_D>2^15-1
      |     f16CC2sc_D=2^15-1;
      |     warning(['Parameter f16CC2sc_D of ' gcb ' exceeds the fixed-point range.']);
      |   end
      |   if f16CC2sc_D<-2^15
      |     f16CC2sc_D=-2^15;
      |     warning(['Parameter f16CC2sc_D of ' gcb ' exceeds the fixed-point range.']);
      |   end
      |   f16CC1sc_Q=round(cc1fq*2^(-u16NShift_Q)*2^15);
      |   if f16CC1sc_Q>2^15-1
      |     f16CC1sc_Q=2^15-1;
      |     warning(['Parameter f16CC1sc_Q of ' gcb ' exceeds the fixed-point range.']);
      |   end
      |   if f16CC1sc_Q<-2^15
      |     f16CC1sc_Q=-2^15;
      |     warning(['Parameter f16CC1sc_Q of ' gcb ' exceeds the fixed-point range.']);
      |   end
      |   f16CC2sc_Q=round(cc2fq*2^(-u16NShift_Q)*2^15);
      |   if f16CC2sc_Q>2^15-1
      |     f16CC2sc_Q=2^15-1;
      |     warning(['Parameter f16CC2sc_Q of ' gcb ' exceeds the fixed-point range.']);
      |   end
      |   if f16CC2sc_Q<-2^15
      |     f16CC2sc_Q=-2^15;
      |     warning(['Parameter f16CC2sc_Q of ' gcb ' exceeds the fixed-point range.']);
      |   end
      |   if isnan(f16CC1sc_D)
      |     if ~strcmp(f16CC1sc_D_bkup,'0')
      |       set_param(gcb,'f16CC1sc_D','0');
      |     end
      |   else
      |     tmps=num2str(f16CC1sc_D);
      |     if ~strcmp(f16CC1sc_D_bkup,tmps)
      |       set_param(gcb,'f16CC1sc_D',tmps);
      |     end
      |   end
      |   if isnan(f16CC2sc_D)
      |     if ~strcmp(f16CC2sc_D_bkup,'0')
      |       set_param(gcb,'f16CC2sc_D','0');
      |     end
      |   else
      |     tmps=num2str(f16CC2sc_D);
      |     if ~strcmp(f16CC2sc_D_bkup,tmps)
      |       set_param(gcb,'f16CC2sc_D',tmps);
      |     end
      |   end
      |   if isnan(u16NShift_D)
      |     if ~strcmp(u16NShift_D_bkup,'0')
      |       set_param(gcb,'u16NShift_D','0');
      |     end
      |   else
      |     tmps=num2str(u16NShift_D);
      |     if ~strcmp(u16NShift_D_bkup,tmps)
      |       set_param(gcb,'u16NShift_D',tmps);
      |     end
      |   end
      |   if isnan(f16CC1sc_Q)
      |     if ~strcmp(f16CC1sc_Q_bkup,'0')
      |       set_param(gcb,'f16CC1sc_Q','0');
      |     end
      |   else
      |     tmps=num2str(f16CC1sc_Q);
      |     if ~strcmp(f16CC1sc_Q_bkup,tmps)
      |       set_param(gcb,'f16CC1sc_Q',tmps);
      |     end
      |   end
      |   if isnan(f16CC2sc_Q)
      |     if ~strcmp(f16CC2sc_Q_bkup,'0')
      |       set_param(gcb,'f16CC2sc_Q','0');
      |     end
      |   else
      |     tmps=num2str(f16CC2sc_Q);
      |     if ~strcmp(f16CC2sc_Q_bkup,tmps)
      |       set_param(gcb,'f16CC2sc_Q',tmps);
      |     end
      |   end
      |   if isnan(u16NShift_Q)
      |     if ~strcmp(u16NShift_Q_bkup,'0')
      |       set_param(gcb,'u16NShift_Q','0');
      |     end
      |   else
      |     tmps=num2str(u16NShift_Q);
      |     if ~strcmp(u16NShift_Q_bkup,tmps)
      |       set_param(gcb,'u16NShift_Q',tmps);
      |     end
      |   end
      | end
      mask Callback if0:
      | autoCalcEn=get_param(gcb,'autoCalcEn');
      | if strcmp(autoCalcEn,'on')
      |   SampleTime=Simulink.data.evalinGlobal(bdroot,get_param(gcb,'SampleTime'));
      |   if (SampleTime==-1)
      |     SampleTime=str2double(get_param(gcb,'SampleTime_1'));
      |   end
      |   f16CC1sc_D_bkup=get_param(gcb,'f16CC1sc_D');
      |   f16CC2sc_D_bkup=get_param(gcb,'f16CC2sc_D');
      |   u16NShift_D_bkup=get_param(gcb,'u16NShift_D');
      |   f16CC1sc_Q_bkup=get_param(gcb,'f16CC1sc_Q');
      |   f16CC2sc_Q_bkup=get_param(gcb,'f16CC2sc_Q');
      |   u16NShift_Q_bkup=get_param(gcb,'u16NShift_Q');
      |   intmethod=get_param(gcb,'intmethod');
      |   if0=Simulink.data.evalinGlobal(bdroot,get_param(gcb,'if0'));
      |   iksi=Simulink.data.evalinGlobal(bdroot,get_param(gcb,'iksi'));
      |   Ld=Simulink.data.evalinGlobal(bdroot,get_param(gcb,'Ld'));
      |   Lq=Simulink.data.evalinGlobal(bdroot,get_param(gcb,'Lq'));
      |   Rs=Simulink.data.evalinGlobal(bdroot,get_param(gcb,'Rs'));
      |   uscale=Simulink.data.evalinGlobal(bdroot,get_param(gcb,'uscale'));
      |   iscale=Simulink.data.evalinGlobal(bdroot,get_param(gcb,'iscale'));
      |   if (if0<=0)
      |     warning('Natural frequency f0 must be positive.');
      |   end
      |   if (iksi<=0)
      |     warning('Current loop attenuation must be positive.');
      |   end
      |   if (iksi>1)
      |     warning('Current loop attenuation must not exceed 1.');
      |   end
      |   if (Ld<=0)
      |     warning('Inductance Ld must be positive.');
      |   end
      |   if (Lq<=0)
      |     warning('Inductance Lq must be positive.');
      |   end
      |   if (Rs<0)
      |     warning('Resistance Rs must be non-negative.');
      |   end
      |   if (uscale<=0)
      |     warning('U_max must be positive.');
      |   end
      |   if (iscale<=0)
      |     warning('I_max must be positive.');
      |   end
      |   w0=6.283185307179586*if0;
      |   pgainD=2.0*iksi*w0*Ld-Rs;
      |   igainD=w0*w0*Ld;
      |   pgainQ=2.0*iksi*w0*Lq-Rs;
      |   igainQ=w0*w0*Lq;
      |   if strcmp(intmethod,'Forward Rectangular')
      |     cc1d=pgainD;
      |     cc2d=-pgainD+igainD*SampleTime;
      |     cc1q=pgainQ;
      |     cc2q=-pgainQ+igainQ*SampleTime;
      |   else
      |     if strcmp(intmethod,'Backward Rectangular')
      |       cc1d=pgainD+igainD*SampleTime;
      |       cc2d=-pgainD;
      |       cc1q=pgainQ+igainQ*SampleTime;
      |       cc2q=-pgainQ;
      |     else
      |       cc1d=pgainD+igainD*SampleTime*0.5;
      |       cc2d=-pgainD+igainD*SampleTime*0.5;
      |       cc1q=pgainQ+igainQ*SampleTime*0.5;
      |       cc2q=-pgainQ+igainQ*SampleTime*0.5;
      |     end
      |   end
      |   cc1fd=cc1d*iscale/uscale;
      |   cc2fd=cc2d*iscale/uscale;
      |   cc1fq=cc1q*iscale/uscale;
      |   cc2fq=cc2q*iscale/uscale;
      |   u16NShift_D=ceil(log2(abs(cc1fd)));
      |   tmpsh=ceil(log2(abs(cc2fd)));
      |   if u16NShift_D<tmpsh
      |     u16NShift_D=tmpsh;
      |   end
      |   if u16NShift_D<0
      |     u16NShift_D=0;
      |   end
      |   if u16NShift_D>15
      |     u16NShift_D=15;
      |     warning(['Parameter u16NShift_D of ' gcb ' exceeds the fixed-point range.']);
      |   end
      |   u16NShift_Q=ceil(log2(abs(cc1fq)));
      |   tmpsh=ceil(log2(abs(cc2fq)));
      |   if u16NShift_Q<tmpsh
      |     u16NShift_Q=tmpsh;
      |   end
      |   if u16NShift_Q<0
      |     u16NShift_Q=0;
      |   end
      |   if u16NShift_Q>15
      |     u16NShift_Q=15;
      |     warning(['Parameter u16NShift_Q of ' gcb ' exceeds the fixed-point range.']);
      |   end
      |   f16CC1sc_D=round(cc1fd*2^(-u16NShift_D)*2^15);
      |   if f16CC1sc_D>2^15-1
      |     f16CC1sc_D=2^15-1;
      |     warning(['Parameter f16CC1sc_D of ' gcb ' exceeds the fixed-point range.']);
      |   end
      |   if f16CC1sc_D<-2^15
      |     f16CC1sc_D=-2^15;
      |     warning(['Parameter f16CC1sc_D of ' gcb ' exceeds the fixed-point range.']);
      |   end
      |   f16CC2sc_D=round(cc2fd*2^(-u16NShift_D)*2^15);
      |   if f16CC2sc_D>2^15-1
      |     f16CC2sc_D=2^15-1;
      |     warning(['Parameter f16CC2sc_D of ' gcb ' exceeds the fixed-point range.']);
      |   end
      |   if f16CC2sc_D<-2^15
      |     f16CC2sc_D=-2^15;
      |     warning(['Parameter f16CC2sc_D of ' gcb ' exceeds the fixed-point range.']);
      |   end
      |   f16CC1sc_Q=round(cc1fq*2^(-u16NShift_Q)*2^15);
      |   if f16CC1sc_Q>2^15-1
      |     f16CC1sc_Q=2^15-1;
      |     warning(['Parameter f16CC1sc_Q of ' gcb ' exceeds the fixed-point range.']);
      |   end
      |   if f16CC1sc_Q<-2^15
      |     f16CC1sc_Q=-2^15;
      |     warning(['Parameter f16CC1sc_Q of ' gcb ' exceeds the fixed-point range.']);
      |   end
      |   f16CC2sc_Q=round(cc2fq*2^(-u16NShift_Q)*2^15);
      |   if f16CC2sc_Q>2^15-1
      |     f16CC2sc_Q=2^15-1;
      |     warning(['Parameter f16CC2sc_Q of ' gcb ' exceeds the fixed-point range.']);
      |   end
      |   if f16CC2sc_Q<-2^15
      |     f16CC2sc_Q=-2^15;
      |     warning(['Parameter f16CC2sc_Q of ' gcb ' exceeds the fixed-point range.']);
      |   end
      |   if isnan(f16CC1sc_D)
      |     if ~strcmp(f16CC1sc_D_bkup,'0')
      |       set_param(gcb,'f16CC1sc_D','0');
      |     end
      |   else
      |     tmps=num2str(f16CC1sc_D);
      |     if ~strcmp(f16CC1sc_D_bkup,tmps)
      |       set_param(gcb,'f16CC1sc_D',tmps);
      |     end
      |   end
      |   if isnan(f16CC2sc_D)
      |     if ~strcmp(f16CC2sc_D_bkup,'0')
      |       set_param(gcb,'f16CC2sc_D','0');
      |     end
      |   else
      |     tmps=num2str(f16CC2sc_D);
      |     if ~strcmp(f16CC2sc_D_bkup,tmps)
      |       set_param(gcb,'f16CC2sc_D',tmps);
      |     end
      |   end
      |   if isnan(u16NShift_D)
      |     if ~strcmp(u16NShift_D_bkup,'0')
      |       set_param(gcb,'u16NShift_D','0');
      |     end
      |   else
      |     tmps=num2str(u16NShift_D);
      |     if ~strcmp(u16NShift_D_bkup,tmps)
      |       set_param(gcb,'u16NShift_D',tmps);
      |     end
      |   end
      |   if isnan(f16CC1sc_Q)
      |     if ~strcmp(f16CC1sc_Q_bkup,'0')
      |       set_param(gcb,'f16CC1sc_Q','0');
      |     end
      |   else
      |     tmps=num2str(f16CC1sc_Q);
      |     if ~strcmp(f16CC1sc_Q_bkup,tmps)
      |       set_param(gcb,'f16CC1sc_Q',tmps);
      |     end
      |   end
      |   if isnan(f16CC2sc_Q)
      |     if ~strcmp(f16CC2sc_Q_bkup,'0')
      |       set_param(gcb,'f16CC2sc_Q','0');
      |     end
      |   else
      |     tmps=num2str(f16CC2sc_Q);
      |     if ~strcmp(f16CC2sc_Q_bkup,tmps)
      |       set_param(gcb,'f16CC2sc_Q',tmps);
      |     end
      |   end
      |   if isnan(u16NShift_Q)
      |     if ~strcmp(u16NShift_Q_bkup,'0')
      |       set_param(gcb,'u16NShift_Q','0');
      |     end
      |   else
      |     tmps=num2str(u16NShift_Q);
      |     if ~strcmp(u16NShift_Q_bkup,tmps)
      |       set_param(gcb,'u16NShift_Q',tmps);
      |     end
      |   end
      | end
      mask Callback iksi:
      | autoCalcEn=get_param(gcb,'autoCalcEn');
      | if strcmp(autoCalcEn,'on')
      |   SampleTime=Simulink.data.evalinGlobal(bdroot,get_param(gcb,'SampleTime'));
      |   if (SampleTime==-1)
      |     SampleTime=str2double(get_param(gcb,'SampleTime_1'));
      |   end
      |   f16CC1sc_D_bkup=get_param(gcb,'f16CC1sc_D');
      |   f16CC2sc_D_bkup=get_param(gcb,'f16CC2sc_D');
      |   u16NShift_D_bkup=get_param(gcb,'u16NShift_D');
      |   f16CC1sc_Q_bkup=get_param(gcb,'f16CC1sc_Q');
      |   f16CC2sc_Q_bkup=get_param(gcb,'f16CC2sc_Q');
      |   u16NShift_Q_bkup=get_param(gcb,'u16NShift_Q');
      |   intmethod=get_param(gcb,'intmethod');
      |   if0=Simulink.data.evalinGlobal(bdroot,get_param(gcb,'if0'));
      |   iksi=Simulink.data.evalinGlobal(bdroot,get_param(gcb,'iksi'));
      |   Ld=Simulink.data.evalinGlobal(bdroot,get_param(gcb,'Ld'));
      |   Lq=Simulink.data.evalinGlobal(bdroot,get_param(gcb,'Lq'));
      |   Rs=Simulink.data.evalinGlobal(bdroot,get_param(gcb,'Rs'));
      |   uscale=Simulink.data.evalinGlobal(bdroot,get_param(gcb,'uscale'));
      |   iscale=Simulink.data.evalinGlobal(bdroot,get_param(gcb,'iscale'));
      |   if (if0<=0)
      |     warning('Natural frequency f0 must be positive.');
      |   end
      |   if (iksi<=0)
      |     warning('Current loop attenuation must be positive.');
      |   end
      |   if (iksi>1)
      |     warning('Current loop attenuation must not exceed 1.');
      |   end
      |   if (Ld<=0)
      |     warning('Inductance Ld must be positive.');
      |   end
      |   if (Lq<=0)
      |     warning('Inductance Lq must be positive.');
      |   end
      |   if (Rs<0)
      |     warning('Resistance Rs must be non-negative.');
      |   end
      |   if (uscale<=0)
      |     warning('U_max must be positive.');
      |   end
      |   if (iscale<=0)
      |     warning('I_max must be positive.');
      |   end
      |   w0=6.283185307179586*if0;
      |   pgainD=2.0*iksi*w0*Ld-Rs;
      |   igainD=w0*w0*Ld;
      |   pgainQ=2.0*iksi*w0*Lq-Rs;
      |   igainQ=w0*w0*Lq;
      |   if strcmp(intmethod,'Forward Rectangular')
      |     cc1d=pgainD;
      |     cc2d=-pgainD+igainD*SampleTime;
      |     cc1q=pgainQ;
      |     cc2q=-pgainQ+igainQ*SampleTime;
      |   else
      |     if strcmp(intmethod,'Backward Rectangular')
      |       cc1d=pgainD+igainD*SampleTime;
      |       cc2d=-pgainD;
      |       cc1q=pgainQ+igainQ*SampleTime;
      |       cc2q=-pgainQ;
      |     else
      |       cc1d=pgainD+igainD*SampleTime*0.5;
      |       cc2d=-pgainD+igainD*SampleTime*0.5;
      |       cc1q=pgainQ+igainQ*SampleTime*0.5;
      |       cc2q=-pgainQ+igainQ*SampleTime*0.5;
      |     end
      |   end
      |   cc1fd=cc1d*iscale/uscale;
      |   cc2fd=cc2d*iscale/uscale;
      |   cc1fq=cc1q*iscale/uscale;
      |   cc2fq=cc2q*iscale/uscale;
      |   u16NShift_D=ceil(log2(abs(cc1fd)));
      |   tmpsh=ceil(log2(abs(cc2fd)));
      |   if u16NShift_D<tmpsh
      |     u16NShift_D=tmpsh;
      |   end
      |   if u16NShift_D<0
      |     u16NShift_D=0;
      |   end
      |   if u16NShift_D>15
      |     u16NShift_D=15;
      |     warning(['Parameter u16NShift_D of ' gcb ' exceeds the fixed-point range.']);
      |   end
      |   u16NShift_Q=ceil(log2(abs(cc1fq)));
      |   tmpsh=ceil(log2(abs(cc2fq)));
      |   if u16NShift_Q<tmpsh
      |     u16NShift_Q=tmpsh;
      |   end
      |   if u16NShift_Q<0
      |     u16NShift_Q=0;
      |   end
      |   if u16NShift_Q>15
      |     u16NShift_Q=15;
      |     warning(['Parameter u16NShift_Q of ' gcb ' exceeds the fixed-point range.']);
      |   end
      |   f16CC1sc_D=round(cc1fd*2^(-u16NShift_D)*2^15);
      |   if f16CC1sc_D>2^15-1
      |     f16CC1sc_D=2^15-1;
      |     warning(['Parameter f16CC1sc_D of ' gcb ' exceeds the fixed-point range.']);
      |   end
      |   if f16CC1sc_D<-2^15
      |     f16CC1sc_D=-2^15;
      |     warning(['Parameter f16CC1sc_D of ' gcb ' exceeds the fixed-point range.']);
      |   end
      |   f16CC2sc_D=round(cc2fd*2^(-u16NShift_D)*2^15);
      |   if f16CC2sc_D>2^15-1
      |     f16CC2sc_D=2^15-1;
      |     warning(['Parameter f16CC2sc_D of ' gcb ' exceeds the fixed-point range.']);
      |   end
      |   if f16CC2sc_D<-2^15
      |     f16CC2sc_D=-2^15;
      |     warning(['Parameter f16CC2sc_D of ' gcb ' exceeds the fixed-point range.']);
      |   end
      |   f16CC1sc_Q=round(cc1fq*2^(-u16NShift_Q)*2^15);
      |   if f16CC1sc_Q>2^15-1
      |     f16CC1sc_Q=2^15-1;
      |     warning(['Parameter f16CC1sc_Q of ' gcb ' exceeds the fixed-point range.']);
      |   end
      |   if f16CC1sc_Q<-2^15
      |     f16CC1sc_Q=-2^15;
      |     warning(['Parameter f16CC1sc_Q of ' gcb ' exceeds the fixed-point range.']);
      |   end
      |   f16CC2sc_Q=round(cc2fq*2^(-u16NShift_Q)*2^15);
      |   if f16CC2sc_Q>2^15-1
      |     f16CC2sc_Q=2^15-1;
      |     warning(['Parameter f16CC2sc_Q of ' gcb ' exceeds the fixed-point range.']);
      |   end
      |   if f16CC2sc_Q<-2^15
      |     f16CC2sc_Q=-2^15;
      |     warning(['Parameter f16CC2sc_Q of ' gcb ' exceeds the fixed-point range.']);
      |   end
      |   if isnan(f16CC1sc_D)
      |     if ~strcmp(f16CC1sc_D_bkup,'0')
      |       set_param(gcb,'f16CC1sc_D','0');
      |     end
      |   else
      |     tmps=num2str(f16CC1sc_D);
      |     if ~strcmp(f16CC1sc_D_bkup,tmps)
      |       set_param(gcb,'f16CC1sc_D',tmps);
      |     end
      |   end
      |   if isnan(f16CC2sc_D)
      |     if ~strcmp(f16CC2sc_D_bkup,'0')
      |       set_param(gcb,'f16CC2sc_D','0');
      |     end
      |   else
      |     tmps=num2str(f16CC2sc_D);
      |     if ~strcmp(f16CC2sc_D_bkup,tmps)
      |       set_param(gcb,'f16CC2sc_D',tmps);
      |     end
      |   end
      |   if isnan(u16NShift_D)
      |     if ~strcmp(u16NShift_D_bkup,'0')
      |       set_param(gcb,'u16NShift_D','0');
      |     end
      |   else
      |     tmps=num2str(u16NShift_D);
      |     if ~strcmp(u16NShift_D_bkup,tmps)
      |       set_param(gcb,'u16NShift_D',tmps);
      |     end
      |   end
      |   if isnan(f16CC1sc_Q)
      |     if ~strcmp(f16CC1sc_Q_bkup,'0')
      |       set_param(gcb,'f16CC1sc_Q','0');
      |     end
      |   else
      |     tmps=num2str(f16CC1sc_Q);
      |     if ~strcmp(f16CC1sc_Q_bkup,tmps)
      |       set_param(gcb,'f16CC1sc_Q',tmps);
      |     end
      |   end
      |   if isnan(f16CC2sc_Q)
      |     if ~strcmp(f16CC2sc_Q_bkup,'0')
      |       set_param(gcb,'f16CC2sc_Q','0');
      |     end
      |   else
      |     tmps=num2str(f16CC2sc_Q);
      |     if ~strcmp(f16CC2sc_Q_bkup,tmps)
      |       set_param(gcb,'f16CC2sc_Q',tmps);
      |     end
      |   end
      |   if isnan(u16NShift_Q)
      |     if ~strcmp(u16NShift_Q_bkup,'0')
      |       set_param(gcb,'u16NShift_Q','0');
      |     end
      |   else
      |     tmps=num2str(u16NShift_Q);
      |     if ~strcmp(u16NShift_Q_bkup,tmps)
      |       set_param(gcb,'u16NShift_Q',tmps);
      |     end
      |   end
      | end
      mask Callback Ld:
      | autoCalcEn=get_param(gcb,'autoCalcEn');
      | if strcmp(autoCalcEn,'on')
      |   SampleTime=Simulink.data.evalinGlobal(bdroot,get_param(gcb,'SampleTime'));
      |   if (SampleTime==-1)
      |     SampleTime=str2double(get_param(gcb,'SampleTime_1'));
      |   end
      |   f16CC1sc_D_bkup=get_param(gcb,'f16CC1sc_D');
      |   f16CC2sc_D_bkup=get_param(gcb,'f16CC2sc_D');
      |   u16NShift_D_bkup=get_param(gcb,'u16NShift_D');
      |   f16CC1sc_Q_bkup=get_param(gcb,'f16CC1sc_Q');
      |   f16CC2sc_Q_bkup=get_param(gcb,'f16CC2sc_Q');
      |   u16NShift_Q_bkup=get_param(gcb,'u16NShift_Q');
      |   intmethod=get_param(gcb,'intmethod');
      |   if0=Simulink.data.evalinGlobal(bdroot,get_param(gcb,'if0'));
      |   iksi=Simulink.data.evalinGlobal(bdroot,get_param(gcb,'iksi'));
      |   Ld=Simulink.data.evalinGlobal(bdroot,get_param(gcb,'Ld'));
      |   Lq=Simulink.data.evalinGlobal(bdroot,get_param(gcb,'Lq'));
      |   Rs=Simulink.data.evalinGlobal(bdroot,get_param(gcb,'Rs'));
      |   uscale=Simulink.data.evalinGlobal(bdroot,get_param(gcb,'uscale'));
      |   iscale=Simulink.data.evalinGlobal(bdroot,get_param(gcb,'iscale'));
      |   if (if0<=0)
      |     warning('Natural frequency f0 must be positive.');
      |   end
      |   if (iksi<=0)
      |     warning('Current loop attenuation must be positive.');
      |   end
      |   if (iksi>1)
      |     warning('Current loop attenuation must not exceed 1.');
      |   end
      |   if (Ld<=0)
      |     warning('Inductance Ld must be positive.');
      |   end
      |   if (Lq<=0)
      |     warning('Inductance Lq must be positive.');
      |   end
      |   if (Rs<0)
      |     warning('Resistance Rs must be non-negative.');
      |   end
      |   if (uscale<=0)
      |     warning('U_max must be positive.');
      |   end
      |   if (iscale<=0)
      |     warning('I_max must be positive.');
      |   end
      |   w0=6.283185307179586*if0;
      |   pgainD=2.0*iksi*w0*Ld-Rs;
      |   igainD=w0*w0*Ld;
      |   pgainQ=2.0*iksi*w0*Lq-Rs;
      |   igainQ=w0*w0*Lq;
      |   if strcmp(intmethod,'Forward Rectangular')
      |     cc1d=pgainD;
      |     cc2d=-pgainD+igainD*SampleTime;
      |     cc1q=pgainQ;
      |     cc2q=-pgainQ+igainQ*SampleTime;
      |   else
      |     if strcmp(intmethod,'Backward Rectangular')
      |       cc1d=pgainD+igainD*SampleTime;
      |       cc2d=-pgainD;
      |       cc1q=pgainQ+igainQ*SampleTime;
      |       cc2q=-pgainQ;
      |     else
      |       cc1d=pgainD+igainD*SampleTime*0.5;
      |       cc2d=-pgainD+igainD*SampleTime*0.5;
      |       cc1q=pgainQ+igainQ*SampleTime*0.5;
      |       cc2q=-pgainQ+igainQ*SampleTime*0.5;
      |     end
      |   end
      |   cc1fd=cc1d*iscale/uscale;
      |   cc2fd=cc2d*iscale/uscale;
      |   cc1fq=cc1q*iscale/uscale;
      |   cc2fq=cc2q*iscale/uscale;
      |   u16NShift_D=ceil(log2(abs(cc1fd)));
      |   tmpsh=ceil(log2(abs(cc2fd)));
      |   if u16NShift_D<tmpsh
      |     u16NShift_D=tmpsh;
      |   end
      |   if u16NShift_D<0
      |     u16NShift_D=0;
      |   end
      |   if u16NShift_D>15
      |     u16NShift_D=15;
      |     warning(['Parameter u16NShift_D of ' gcb ' exceeds the fixed-point range.']);
      |   end
      |   u16NShift_Q=ceil(log2(abs(cc1fq)));
      |   tmpsh=ceil(log2(abs(cc2fq)));
      |   if u16NShift_Q<tmpsh
      |     u16NShift_Q=tmpsh;
      |   end
      |   if u16NShift_Q<0
      |     u16NShift_Q=0;
      |   end
      |   if u16NShift_Q>15
      |     u16NShift_Q=15;
      |     warning(['Parameter u16NShift_Q of ' gcb ' exceeds the fixed-point range.']);
      |   end
      |   f16CC1sc_D=round(cc1fd*2^(-u16NShift_D)*2^15);
      |   if f16CC1sc_D>2^15-1
      |     f16CC1sc_D=2^15-1;
      |     warning(['Parameter f16CC1sc_D of ' gcb ' exceeds the fixed-point range.']);
      |   end
      |   if f16CC1sc_D<-2^15
      |     f16CC1sc_D=-2^15;
      |     warning(['Parameter f16CC1sc_D of ' gcb ' exceeds the fixed-point range.']);
      |   end
      |   f16CC2sc_D=round(cc2fd*2^(-u16NShift_D)*2^15);
      |   if f16CC2sc_D>2^15-1
      |     f16CC2sc_D=2^15-1;
      |     warning(['Parameter f16CC2sc_D of ' gcb ' exceeds the fixed-point range.']);
      |   end
      |   if f16CC2sc_D<-2^15
      |     f16CC2sc_D=-2^15;
      |     warning(['Parameter f16CC2sc_D of ' gcb ' exceeds the fixed-point range.']);
      |   end
      |   f16CC1sc_Q=round(cc1fq*2^(-u16NShift_Q)*2^15);
      |   if f16CC1sc_Q>2^15-1
      |     f16CC1sc_Q=2^15-1;
      |     warning(['Parameter f16CC1sc_Q of ' gcb ' exceeds the fixed-point range.']);
      |   end
      |   if f16CC1sc_Q<-2^15
      |     f16CC1sc_Q=-2^15;
      |     warning(['Parameter f16CC1sc_Q of ' gcb ' exceeds the fixed-point range.']);
      |   end
      |   f16CC2sc_Q=round(cc2fq*2^(-u16NShift_Q)*2^15);
      |   if f16CC2sc_Q>2^15-1
      |     f16CC2sc_Q=2^15-1;
      |     warning(['Parameter f16CC2sc_Q of ' gcb ' exceeds the fixed-point range.']);
      |   end
      |   if f16CC2sc_Q<-2^15
      |     f16CC2sc_Q=-2^15;
      |     warning(['Parameter f16CC2sc_Q of ' gcb ' exceeds the fixed-point range.']);
      |   end
      |   if isnan(f16CC1sc_D)
      |     if ~strcmp(f16CC1sc_D_bkup,'0')
      |       set_param(gcb,'f16CC1sc_D','0');
      |     end
      |   else
      |     tmps=num2str(f16CC1sc_D);
      |     if ~strcmp(f16CC1sc_D_bkup,tmps)
      |       set_param(gcb,'f16CC1sc_D',tmps);
      |     end
      |   end
      |   if isnan(f16CC2sc_D)
      |     if ~strcmp(f16CC2sc_D_bkup,'0')
      |       set_param(gcb,'f16CC2sc_D','0');
      |     end
      |   else
      |     tmps=num2str(f16CC2sc_D);
      |     if ~strcmp(f16CC2sc_D_bkup,tmps)
      |       set_param(gcb,'f16CC2sc_D',tmps);
      |     end
      |   end
      |   if isnan(u16NShift_D)
      |     if ~strcmp(u16NShift_D_bkup,'0')
      |       set_param(gcb,'u16NShift_D','0');
      |     end
      |   else
      |     tmps=num2str(u16NShift_D);
      |     if ~strcmp(u16NShift_D_bkup,tmps)
      |       set_param(gcb,'u16NShift_D',tmps);
      |     end
      |   end
      |   if isnan(f16CC1sc_Q)
      |     if ~strcmp(f16CC1sc_Q_bkup,'0')
      |       set_param(gcb,'f16CC1sc_Q','0');
      |     end
      |   else
      |     tmps=num2str(f16CC1sc_Q);
      |     if ~strcmp(f16CC1sc_Q_bkup,tmps)
      |       set_param(gcb,'f16CC1sc_Q',tmps);
      |     end
      |   end
      |   if isnan(f16CC2sc_Q)
      |     if ~strcmp(f16CC2sc_Q_bkup,'0')
      |       set_param(gcb,'f16CC2sc_Q','0');
      |     end
      |   else
      |     tmps=num2str(f16CC2sc_Q);
      |     if ~strcmp(f16CC2sc_Q_bkup,tmps)
      |       set_param(gcb,'f16CC2sc_Q',tmps);
      |     end
      |   end
      |   if isnan(u16NShift_Q)
      |     if ~strcmp(u16NShift_Q_bkup,'0')
      |       set_param(gcb,'u16NShift_Q','0');
      |     end
      |   else
      |     tmps=num2str(u16NShift_Q);
      |     if ~strcmp(u16NShift_Q_bkup,tmps)
      |       set_param(gcb,'u16NShift_Q',tmps);
      |     end
      |   end
      | end
      mask Callback Lq:
      | autoCalcEn=get_param(gcb,'autoCalcEn');
      | if strcmp(autoCalcEn,'on')
      |   SampleTime=Simulink.data.evalinGlobal(bdroot,get_param(gcb,'SampleTime'));
      |   if (SampleTime==-1)
      |     SampleTime=str2double(get_param(gcb,'SampleTime_1'));
      |   end
      |   f16CC1sc_D_bkup=get_param(gcb,'f16CC1sc_D');
      |   f16CC2sc_D_bkup=get_param(gcb,'f16CC2sc_D');
      |   u16NShift_D_bkup=get_param(gcb,'u16NShift_D');
      |   f16CC1sc_Q_bkup=get_param(gcb,'f16CC1sc_Q');
      |   f16CC2sc_Q_bkup=get_param(gcb,'f16CC2sc_Q');
      |   u16NShift_Q_bkup=get_param(gcb,'u16NShift_Q');
      |   intmethod=get_param(gcb,'intmethod');
      |   if0=Simulink.data.evalinGlobal(bdroot,get_param(gcb,'if0'));
      |   iksi=Simulink.data.evalinGlobal(bdroot,get_param(gcb,'iksi'));
      |   Ld=Simulink.data.evalinGlobal(bdroot,get_param(gcb,'Ld'));
      |   Lq=Simulink.data.evalinGlobal(bdroot,get_param(gcb,'Lq'));
      |   Rs=Simulink.data.evalinGlobal(bdroot,get_param(gcb,'Rs'));
      |   uscale=Simulink.data.evalinGlobal(bdroot,get_param(gcb,'uscale'));
      |   iscale=Simulink.data.evalinGlobal(bdroot,get_param(gcb,'iscale'));
      |   if (if0<=0)
      |     warning('Natural frequency f0 must be positive.');
      |   end
      |   if (iksi<=0)
      |     warning('Current loop attenuation must be positive.');
      |   end
      |   if (iksi>1)
      |     warning('Current loop attenuation must not exceed 1.');
      |   end
      |   if (Ld<=0)
      |     warning('Inductance Ld must be positive.');
      |   end
      |   if (Lq<=0)
      |     warning('Inductance Lq must be positive.');
      |   end
      |   if (Rs<0)
      |     warning('Resistance Rs must be non-negative.');
      |   end
      |   if (uscale<=0)
      |     warning('U_max must be positive.');
      |   end
      |   if (iscale<=0)
      |     warning('I_max must be positive.');
      |   end
      |   w0=6.283185307179586*if0;
      |   pgainD=2.0*iksi*w0*Ld-Rs;
      |   igainD=w0*w0*Ld;
      |   pgainQ=2.0*iksi*w0*Lq-Rs;
      |   igainQ=w0*w0*Lq;
      |   if strcmp(intmethod,'Forward Rectangular')
      |     cc1d=pgainD;
      |     cc2d=-pgainD+igainD*SampleTime;
      |     cc1q=pgainQ;
      |     cc2q=-pgainQ+igainQ*SampleTime;
      |   else
      |     if strcmp(intmethod,'Backward Rectangular')
      |       cc1d=pgainD+igainD*SampleTime;
      |       cc2d=-pgainD;
      |       cc1q=pgainQ+igainQ*SampleTime;
      |       cc2q=-pgainQ;
      |     else
      |       cc1d=pgainD+igainD*SampleTime*0.5;
      |       cc2d=-pgainD+igainD*SampleTime*0.5;
      |       cc1q=pgainQ+igainQ*SampleTime*0.5;
      |       cc2q=-pgainQ+igainQ*SampleTime*0.5;
      |     end
      |   end
      |   cc1fd=cc1d*iscale/uscale;
      |   cc2fd=cc2d*iscale/uscale;
      |   cc1fq=cc1q*iscale/uscale;
      |   cc2fq=cc2q*iscale/uscale;
      |   u16NShift_D=ceil(log2(abs(cc1fd)));
      |   tmpsh=ceil(log2(abs(cc2fd)));
      |   if u16NShift_D<tmpsh
      |     u16NShift_D=tmpsh;
      |   end
      |   if u16NShift_D<0
      |     u16NShift_D=0;
      |   end
      |   if u16NShift_D>15
      |     u16NShift_D=15;
      |     warning(['Parameter u16NShift_D of ' gcb ' exceeds the fixed-point range.']);
      |   end
      |   u16NShift_Q=ceil(log2(abs(cc1fq)));
      |   tmpsh=ceil(log2(abs(cc2fq)));
      |   if u16NShift_Q<tmpsh
      |     u16NShift_Q=tmpsh;
      |   end
      |   if u16NShift_Q<0
      |     u16NShift_Q=0;
      |   end
      |   if u16NShift_Q>15
      |     u16NShift_Q=15;
      |     warning(['Parameter u16NShift_Q of ' gcb ' exceeds the fixed-point range.']);
      |   end
      |   f16CC1sc_D=round(cc1fd*2^(-u16NShift_D)*2^15);
      |   if f16CC1sc_D>2^15-1
      |     f16CC1sc_D=2^15-1;
      |     warning(['Parameter f16CC1sc_D of ' gcb ' exceeds the fixed-point range.']);
      |   end
      |   if f16CC1sc_D<-2^15
      |     f16CC1sc_D=-2^15;
      |     warning(['Parameter f16CC1sc_D of ' gcb ' exceeds the fixed-point range.']);
      |   end
      |   f16CC2sc_D=round(cc2fd*2^(-u16NShift_D)*2^15);
      |   if f16CC2sc_D>2^15-1
      |     f16CC2sc_D=2^15-1;
      |     warning(['Parameter f16CC2sc_D of ' gcb ' exceeds the fixed-point range.']);
      |   end
      |   if f16CC2sc_D<-2^15
      |     f16CC2sc_D=-2^15;
      |     warning(['Parameter f16CC2sc_D of ' gcb ' exceeds the fixed-point range.']);
      |   end
      |   f16CC1sc_Q=round(cc1fq*2^(-u16NShift_Q)*2^15);
      |   if f16CC1sc_Q>2^15-1
      |     f16CC1sc_Q=2^15-1;
      |     warning(['Parameter f16CC1sc_Q of ' gcb ' exceeds the fixed-point range.']);
      |   end
      |   if f16CC1sc_Q<-2^15
      |     f16CC1sc_Q=-2^15;
      |     warning(['Parameter f16CC1sc_Q of ' gcb ' exceeds the fixed-point range.']);
      |   end
      |   f16CC2sc_Q=round(cc2fq*2^(-u16NShift_Q)*2^15);
      |   if f16CC2sc_Q>2^15-1
      |     f16CC2sc_Q=2^15-1;
      |     warning(['Parameter f16CC2sc_Q of ' gcb ' exceeds the fixed-point range.']);
      |   end
      |   if f16CC2sc_Q<-2^15
      |     f16CC2sc_Q=-2^15;
      |     warning(['Parameter f16CC2sc_Q of ' gcb ' exceeds the fixed-point range.']);
      |   end
      |   if isnan(f16CC1sc_D)
      |     if ~strcmp(f16CC1sc_D_bkup,'0')
      |       set_param(gcb,'f16CC1sc_D','0');
      |     end
      |   else
      |     tmps=num2str(f16CC1sc_D);
      |     if ~strcmp(f16CC1sc_D_bkup,tmps)
      |       set_param(gcb,'f16CC1sc_D',tmps);
      |     end
      |   end
      |   if isnan(f16CC2sc_D)
      |     if ~strcmp(f16CC2sc_D_bkup,'0')
      |       set_param(gcb,'f16CC2sc_D','0');
      |     end
      |   else
      |     tmps=num2str(f16CC2sc_D);
      |     if ~strcmp(f16CC2sc_D_bkup,tmps)
      |       set_param(gcb,'f16CC2sc_D',tmps);
      |     end
      |   end
      |   if isnan(u16NShift_D)
      |     if ~strcmp(u16NShift_D_bkup,'0')
      |       set_param(gcb,'u16NShift_D','0');
      |     end
      |   else
      |     tmps=num2str(u16NShift_D);
      |     if ~strcmp(u16NShift_D_bkup,tmps)
      |       set_param(gcb,'u16NShift_D',tmps);
      |     end
      |   end
      |   if isnan(f16CC1sc_Q)
      |     if ~strcmp(f16CC1sc_Q_bkup,'0')
      |       set_param(gcb,'f16CC1sc_Q','0');
      |     end
      |   else
      |     tmps=num2str(f16CC1sc_Q);
      |     if ~strcmp(f16CC1sc_Q_bkup,tmps)
      |       set_param(gcb,'f16CC1sc_Q',tmps);
      |     end
      |   end
      |   if isnan(f16CC2sc_Q)
      |     if ~strcmp(f16CC2sc_Q_bkup,'0')
      |       set_param(gcb,'f16CC2sc_Q','0');
      |     end
      |   else
      |     tmps=num2str(f16CC2sc_Q);
      |     if ~strcmp(f16CC2sc_Q_bkup,tmps)
      |       set_param(gcb,'f16CC2sc_Q',tmps);
      |     end
      |   end
      |   if isnan(u16NShift_Q)
      |     if ~strcmp(u16NShift_Q_bkup,'0')
      |       set_param(gcb,'u16NShift_Q','0');
      |     end
      |   else
      |     tmps=num2str(u16NShift_Q);
      |     if ~strcmp(u16NShift_Q_bkup,tmps)
      |       set_param(gcb,'u16NShift_Q',tmps);
      |     end
      |   end
      | end
      mask Callback Rs:
      | autoCalcEn=get_param(gcb,'autoCalcEn');
      | if strcmp(autoCalcEn,'on')
      |   SampleTime=Simulink.data.evalinGlobal(bdroot,get_param(gcb,'SampleTime'));
      |   if (SampleTime==-1)
      |     SampleTime=str2double(get_param(gcb,'SampleTime_1'));
      |   end
      |   f16CC1sc_D_bkup=get_param(gcb,'f16CC1sc_D');
      |   f16CC2sc_D_bkup=get_param(gcb,'f16CC2sc_D');
      |   u16NShift_D_bkup=get_param(gcb,'u16NShift_D');
      |   f16CC1sc_Q_bkup=get_param(gcb,'f16CC1sc_Q');
      |   f16CC2sc_Q_bkup=get_param(gcb,'f16CC2sc_Q');
      |   u16NShift_Q_bkup=get_param(gcb,'u16NShift_Q');
      |   intmethod=get_param(gcb,'intmethod');
      |   if0=Simulink.data.evalinGlobal(bdroot,get_param(gcb,'if0'));
      |   iksi=Simulink.data.evalinGlobal(bdroot,get_param(gcb,'iksi'));
      |   Ld=Simulink.data.evalinGlobal(bdroot,get_param(gcb,'Ld'));
      |   Lq=Simulink.data.evalinGlobal(bdroot,get_param(gcb,'Lq'));
      |   Rs=Simulink.data.evalinGlobal(bdroot,get_param(gcb,'Rs'));
      |   uscale=Simulink.data.evalinGlobal(bdroot,get_param(gcb,'uscale'));
      |   iscale=Simulink.data.evalinGlobal(bdroot,get_param(gcb,'iscale'));
      |   if (if0<=0)
      |     warning('Natural frequency f0 must be positive.');
      |   end
      |   if (iksi<=0)
      |     warning('Current loop attenuation must be positive.');
      |   end
      |   if (iksi>1)
      |     warning('Current loop attenuation must not exceed 1.');
      |   end
      |   if (Ld<=0)
      |     warning('Inductance Ld must be positive.');
      |   end
      |   if (Lq<=0)
      |     warning('Inductance Lq must be positive.');
      |   end
      |   if (Rs<0)
      |     warning('Resistance Rs must be non-negative.');
      |   end
      |   if (uscale<=0)
      |     warning('U_max must be positive.');
      |   end
      |   if (iscale<=0)
      |     warning('I_max must be positive.');
      |   end
      |   w0=6.283185307179586*if0;
      |   pgainD=2.0*iksi*w0*Ld-Rs;
      |   igainD=w0*w0*Ld;
      |   pgainQ=2.0*iksi*w0*Lq-Rs;
      |   igainQ=w0*w0*Lq;
      |   if strcmp(intmethod,'Forward Rectangular')
      |     cc1d=pgainD;
      |     cc2d=-pgainD+igainD*SampleTime;
      |     cc1q=pgainQ;
      |     cc2q=-pgainQ+igainQ*SampleTime;
      |   else
      |     if strcmp(intmethod,'Backward Rectangular')
      |       cc1d=pgainD+igainD*SampleTime;
      |       cc2d=-pgainD;
      |       cc1q=pgainQ+igainQ*SampleTime;
      |       cc2q=-pgainQ;
      |     else
      |       cc1d=pgainD+igainD*SampleTime*0.5;
      |       cc2d=-pgainD+igainD*SampleTime*0.5;
      |       cc1q=pgainQ+igainQ*SampleTime*0.5;
      |       cc2q=-pgainQ+igainQ*SampleTime*0.5;
      |     end
      |   end
      |   cc1fd=cc1d*iscale/uscale;
      |   cc2fd=cc2d*iscale/uscale;
      |   cc1fq=cc1q*iscale/uscale;
      |   cc2fq=cc2q*iscale/uscale;
      |   u16NShift_D=ceil(log2(abs(cc1fd)));
      |   tmpsh=ceil(log2(abs(cc2fd)));
      |   if u16NShift_D<tmpsh
      |     u16NShift_D=tmpsh;
      |   end
      |   if u16NShift_D<0
      |     u16NShift_D=0;
      |   end
      |   if u16NShift_D>15
      |     u16NShift_D=15;
      |     warning(['Parameter u16NShift_D of ' gcb ' exceeds the fixed-point range.']);
      |   end
      |   u16NShift_Q=ceil(log2(abs(cc1fq)));
      |   tmpsh=ceil(log2(abs(cc2fq)));
      |   if u16NShift_Q<tmpsh
      |     u16NShift_Q=tmpsh;
      |   end
      |   if u16NShift_Q<0
      |     u16NShift_Q=0;
      |   end
      |   if u16NShift_Q>15
      |     u16NShift_Q=15;
      |     warning(['Parameter u16NShift_Q of ' gcb ' exceeds the fixed-point range.']);
      |   end
      |   f16CC1sc_D=round(cc1fd*2^(-u16NShift_D)*2^15);
      |   if f16CC1sc_D>2^15-1
      |     f16CC1sc_D=2^15-1;
      |     warning(['Parameter f16CC1sc_D of ' gcb ' exceeds the fixed-point range.']);
      |   end
      |   if f16CC1sc_D<-2^15
      |     f16CC1sc_D=-2^15;
      |     warning(['Parameter f16CC1sc_D of ' gcb ' exceeds the fixed-point range.']);
      |   end
      |   f16CC2sc_D=round(cc2fd*2^(-u16NShift_D)*2^15);
      |   if f16CC2sc_D>2^15-1
      |     f16CC2sc_D=2^15-1;
      |     warning(['Parameter f16CC2sc_D of ' gcb ' exceeds the fixed-point range.']);
      |   end
      |   if f16CC2sc_D<-2^15
      |     f16CC2sc_D=-2^15;
      |     warning(['Parameter f16CC2sc_D of ' gcb ' exceeds the fixed-point range.']);
      |   end
      |   f16CC1sc_Q=round(cc1fq*2^(-u16NShift_Q)*2^15);
      |   if f16CC1sc_Q>2^15-1
      |     f16CC1sc_Q=2^15-1;
      |     warning(['Parameter f16CC1sc_Q of ' gcb ' exceeds the fixed-point range.']);
      |   end
      |   if f16CC1sc_Q<-2^15
      |     f16CC1sc_Q=-2^15;
      |     warning(['Parameter f16CC1sc_Q of ' gcb ' exceeds the fixed-point range.']);
      |   end
      |   f16CC2sc_Q=round(cc2fq*2^(-u16NShift_Q)*2^15);
      |   if f16CC2sc_Q>2^15-1
      |     f16CC2sc_Q=2^15-1;
      |     warning(['Parameter f16CC2sc_Q of ' gcb ' exceeds the fixed-point range.']);
      |   end
      |   if f16CC2sc_Q<-2^15
      |     f16CC2sc_Q=-2^15;
      |     warning(['Parameter f16CC2sc_Q of ' gcb ' exceeds the fixed-point range.']);
      |   end
      |   if isnan(f16CC1sc_D)
      |     if ~strcmp(f16CC1sc_D_bkup,'0')
      |       set_param(gcb,'f16CC1sc_D','0');
      |     end
      |   else
      |     tmps=num2str(f16CC1sc_D);
      |     if ~strcmp(f16CC1sc_D_bkup,tmps)
      |       set_param(gcb,'f16CC1sc_D',tmps);
      |     end
      |   end
      |   if isnan(f16CC2sc_D)
      |     if ~strcmp(f16CC2sc_D_bkup,'0')
      |       set_param(gcb,'f16CC2sc_D','0');
      |     end
      |   else
      |     tmps=num2str(f16CC2sc_D);
      |     if ~strcmp(f16CC2sc_D_bkup,tmps)
      |       set_param(gcb,'f16CC2sc_D',tmps);
      |     end
      |   end
      |   if isnan(u16NShift_D)
      |     if ~strcmp(u16NShift_D_bkup,'0')
      |       set_param(gcb,'u16NShift_D','0');
      |     end
      |   else
      |     tmps=num2str(u16NShift_D);
      |     if ~strcmp(u16NShift_D_bkup,tmps)
      |       set_param(gcb,'u16NShift_D',tmps);
      |     end
      |   end
      |   if isnan(f16CC1sc_Q)
      |     if ~strcmp(f16CC1sc_Q_bkup,'0')
      |       set_param(gcb,'f16CC1sc_Q','0');
      |     end
      |   else
      |     tmps=num2str(f16CC1sc_Q);
      |     if ~strcmp(f16CC1sc_Q_bkup,tmps)
      |       set_param(gcb,'f16CC1sc_Q',tmps);
      |     end
      |   end
      |   if isnan(f16CC2sc_Q)
      |     if ~strcmp(f16CC2sc_Q_bkup,'0')
      |       set_param(gcb,'f16CC2sc_Q','0');
      |     end
      |   else
      |     tmps=num2str(f16CC2sc_Q);
      |     if ~strcmp(f16CC2sc_Q_bkup,tmps)
      |       set_param(gcb,'f16CC2sc_Q',tmps);
      |     end
      |   end
      |   if isnan(u16NShift_Q)
      |     if ~strcmp(u16NShift_Q_bkup,'0')
      |       set_param(gcb,'u16NShift_Q','0');
      |     end
      |   else
      |     tmps=num2str(u16NShift_Q);
      |     if ~strcmp(u16NShift_Q_bkup,tmps)
      |       set_param(gcb,'u16NShift_Q',tmps);
      |     end
      |   end
      | end
      mask Callback uscale:
      | autoCalcEn=get_param(gcb,'autoCalcEn');
      | if strcmp(autoCalcEn,'on')
      |   SampleTime=Simulink.data.evalinGlobal(bdroot,get_param(gcb,'SampleTime'));
      |   if (SampleTime==-1)
      |     SampleTime=str2double(get_param(gcb,'SampleTime_1'));
      |   end
      |   f16CC1sc_D_bkup=get_param(gcb,'f16CC1sc_D');
      |   f16CC2sc_D_bkup=get_param(gcb,'f16CC2sc_D');
      |   u16NShift_D_bkup=get_param(gcb,'u16NShift_D');
      |   f16CC1sc_Q_bkup=get_param(gcb,'f16CC1sc_Q');
      |   f16CC2sc_Q_bkup=get_param(gcb,'f16CC2sc_Q');
      |   u16NShift_Q_bkup=get_param(gcb,'u16NShift_Q');
      |   intmethod=get_param(gcb,'intmethod');
      |   if0=Simulink.data.evalinGlobal(bdroot,get_param(gcb,'if0'));
      |   iksi=Simulink.data.evalinGlobal(bdroot,get_param(gcb,'iksi'));
      |   Ld=Simulink.data.evalinGlobal(bdroot,get_param(gcb,'Ld'));
      |   Lq=Simulink.data.evalinGlobal(bdroot,get_param(gcb,'Lq'));
      |   Rs=Simulink.data.evalinGlobal(bdroot,get_param(gcb,'Rs'));
      |   uscale=Simulink.data.evalinGlobal(bdroot,get_param(gcb,'uscale'));
      |   iscale=Simulink.data.evalinGlobal(bdroot,get_param(gcb,'iscale'));
      |   if (if0<=0)
      |     warning('Natural frequency f0 must be positive.');
      |   end
      |   if (iksi<=0)
      |     warning('Current loop attenuation must be positive.');
      |   end
      |   if (iksi>1)
      |     warning('Current loop attenuation must not exceed 1.');
      |   end
      |   if (Ld<=0)
      |     warning('Inductance Ld must be positive.');
      |   end
      |   if (Lq<=0)
      |     warning('Inductance Lq must be positive.');
      |   end
      |   if (Rs<0)
      |     warning('Resistance Rs must be non-negative.');
      |   end
      |   if (uscale<=0)
      |     warning('U_max must be positive.');
      |   end
      |   if (iscale<=0)
      |     warning('I_max must be positive.');
      |   end
      |   w0=6.283185307179586*if0;
      |   pgainD=2.0*iksi*w0*Ld-Rs;
      |   igainD=w0*w0*Ld;
      |   pgainQ=2.0*iksi*w0*Lq-Rs;
      |   igainQ=w0*w0*Lq;
      |   if strcmp(intmethod,'Forward Rectangular')
      |     cc1d=pgainD;
      |     cc2d=-pgainD+igainD*SampleTime;
      |     cc1q=pgainQ;
      |     cc2q=-pgainQ+igainQ*SampleTime;
      |   else
      |     if strcmp(intmethod,'Backward Rectangular')
      |       cc1d=pgainD+igainD*SampleTime;
      |       cc2d=-pgainD;
      |       cc1q=pgainQ+igainQ*SampleTime;
      |       cc2q=-pgainQ;
      |     else
      |       cc1d=pgainD+igainD*SampleTime*0.5;
      |       cc2d=-pgainD+igainD*SampleTime*0.5;
      |       cc1q=pgainQ+igainQ*SampleTime*0.5;
      |       cc2q=-pgainQ+igainQ*SampleTime*0.5;
      |     end
      |   end
      |   cc1fd=cc1d*iscale/uscale;
      |   cc2fd=cc2d*iscale/uscale;
      |   cc1fq=cc1q*iscale/uscale;
      |   cc2fq=cc2q*iscale/uscale;
      |   u16NShift_D=ceil(log2(abs(cc1fd)));
      |   tmpsh=ceil(log2(abs(cc2fd)));
      |   if u16NShift_D<tmpsh
      |     u16NShift_D=tmpsh;
      |   end
      |   if u16NShift_D<0
      |     u16NShift_D=0;
      |   end
      |   if u16NShift_D>15
      |     u16NShift_D=15;
      |     warning(['Parameter u16NShift_D of ' gcb ' exceeds the fixed-point range.']);
      |   end
      |   u16NShift_Q=ceil(log2(abs(cc1fq)));
      |   tmpsh=ceil(log2(abs(cc2fq)));
      |   if u16NShift_Q<tmpsh
      |     u16NShift_Q=tmpsh;
      |   end
      |   if u16NShift_Q<0
      |     u16NShift_Q=0;
      |   end
      |   if u16NShift_Q>15
